simulink model "c00002M_harness"  (R2018a)
settings: Solver=ode3  StartTime=0.0  StopTime=10.0  RelTol=1e-3  EnableMultiTasking=on
undefined symbols (not defined in the file): b, DiscIntNeverNeededParam, J, K, L, PosMinimaW3, PosMinimaW4, R, sigbuilder_block
(part 1 of 75)
settings Model: Creator=aarrieta  LastModifiedBy=umarkiegi
settings DataIOCC: LimitDataPoints=on  SaveFormat=Array
settings OptimizationCC: LifeSpan=inf
settings DebuggingCC: UnderspecifiedInitializationDetection=Classic  MergeDetectMultiDrivingBlocksExec=none  SolverPrmCheckMsg=warning  StateNameClashWarn=warning  SFUnexpectedBacktrackingDiag=warning  SFNoUnconditionalDefaultTransitionDiag=warning  SFExecutionAtInitializationDiag=none
settings HardwareCC: ProdBitPerPointer=32  ProdBitPerSizeT=32  ProdBitPerPtrDiffT=32  ProdLargestAtomicFloat=None  ProdIntDivRoundTo=Undefined  ProdEndianess=Unspecified  ProdWordSize=32  ProdHWDeviceType=32-bit Generic
settings ModelReferenceCC: PropagateSignalLabelsOutOfModel=off
settings CodeAppCC: StateflowObjectComments=on
settings GRTTargetCC: TargetLangStandard=C89/C90 (ANSI)  GeneratePreprocessorConditionals=Disable all
settings ConfigComp: CovMetricSettings=dw  CovHtmlReporting=on  CovSaveCumulativeToWorkspaceVar=on  CovSaveSingleToWorkspaceVar=on  CovExternalEMLEnable=off  DVMaxTestCaseSteps=20  DVTestSuiteOptimization=CombinedObjectives (Nonlinear Extended)  DVDetectFloatOverflow=off

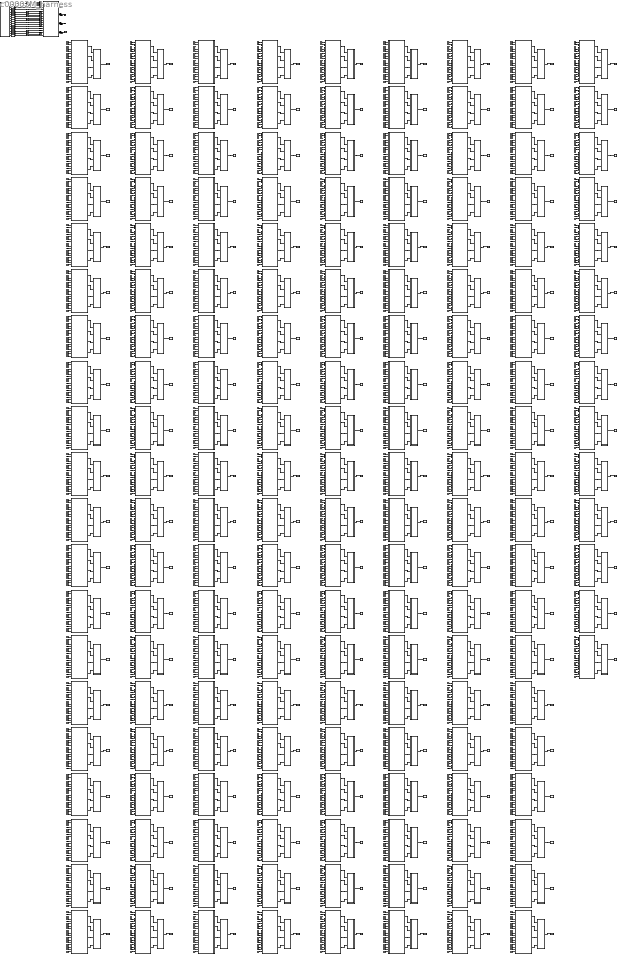
== system c00002M_harness ==
  CPSUT : Subsystem
  Eval : Subsystem
  Eval1 : Subsystem
  Eval10 : Subsystem
  Eval100 : Subsystem
  Eval101 : Subsystem
  Eval102 : Subsystem
  Eval103 : Subsystem
  Eval104 : Subsystem
  Eval105 : Subsystem
  Eval106 : Subsystem
  Eval107 : Subsystem
  Eval108 : Subsystem
  Eval109 : Subsystem
  Eval11 : Subsystem
  Eval110 : Subsystem
  Eval111 : Subsystem
  Eval112 : Subsystem
  Eval113 : Subsystem
  Eval114 : Subsystem
  Eval115 : Subsystem
  Eval116 : Subsystem
  Eval117 : Subsystem
  Eval118 : Subsystem
  Eval119 : Subsystem
  Eval12 : Subsystem
  Eval120 : Subsystem
  Eval121 : Subsystem
  Eval122 : Subsystem
  Eval123 : Subsystem
  Eval124 : Subsystem
  Eval125 : Subsystem
  Eval126 : Subsystem
  Eval127 : Subsystem
  Eval128 : Subsystem
  Eval129 : Subsystem
  Eval13 : Subsystem
  Eval130 : Subsystem
  Eval131 : Subsystem
  Eval132 : Subsystem
  Eval133 : Subsystem
  Eval134 : Subsystem
  Eval135 : Subsystem
  Eval136 : Subsystem
  Eval137 : Subsystem
  Eval138 : Subsystem
  Eval139 : Subsystem
  Eval14 : Subsystem
  Eval140 : Subsystem
  Eval141 : Subsystem
  Eval142 : Subsystem
  Eval143 : Subsystem
  Eval144 : Subsystem
  Eval145 : Subsystem
  Eval146 : Subsystem
  Eval147 : Subsystem
  Eval148 : Subsystem
  Eval149 : Subsystem
  Eval15 : Subsystem
  Eval150 : Subsystem
  Eval151 : Subsystem
  Eval152 : Subsystem
  Eval153 : Subsystem
  Eval154 : Subsystem
  Eval155 : Subsystem
  Eval156 : Subsystem
  Eval157 : Subsystem
  Eval158 : Subsystem
  Eval159 : Subsystem
  Eval16 : Subsystem
  Eval160 : Subsystem
  Eval161 : Subsystem
  Eval162 : Subsystem
  Eval163 : Subsystem
  Eval164 : Subsystem
  Eval165 : Subsystem
  Eval166 : Subsystem
  Eval167 : Subsystem
  Eval168 : Subsystem
  Eval169 : Subsystem
  Eval17 : Subsystem
  Eval170 : Subsystem
  Eval171 : Subsystem
  Eval172 : Subsystem
  Eval173 : Subsystem
  Eval18 : Subsystem
  Eval19 : Subsystem
  Eval2 : Subsystem
  Eval20 : Subsystem
  Eval21 : Subsystem
  Eval22 : Subsystem
  Eval23 : Subsystem
  Eval24 : Subsystem
  Eval25 : Subsystem
  Eval26 : Subsystem
  Eval27 : Subsystem
  Eval28 : Subsystem
  Eval29 : Subsystem
  Eval3 : Subsystem
  Eval30 : Subsystem
  Eval31 : Subsystem
  Eval32 : Subsystem
  Eval33 : Subsystem
  Eval34 : Subsystem
  Eval35 : Subsystem
  Eval36 : Subsystem
  Eval37 : Subsystem
  Eval38 : Subsystem
  Eval39 : Subsystem
  Eval4 : Subsystem
  Eval40 : Subsystem
  Eval41 : Subsystem
  Eval42 : Subsystem
  Eval43 : Subsystem
  Eval44 : Subsystem
  Eval45 : Subsystem
  Eval46 : Subsystem
  Eval47 : Subsystem
  Eval48 : Subsystem
  Eval49 : Subsystem
  Eval5 : Subsystem
  Eval50 : Subsystem
  Eval51 : Subsystem
  Eval52 : Subsystem
  Eval53 : Subsystem
  Eval54 : Subsystem
  Eval55 : Subsystem
  Eval56 : Subsystem
  Eval57 : Subsystem
  Eval58 : Subsystem
  Eval59 : Subsystem
  Eval6 : Subsystem
  Eval60 : Subsystem
  Eval61 : Subsystem
  Eval62 : Subsystem
  Eval63 : Subsystem
  Eval64 : Subsystem
  Eval65 : Subsystem
  Eval66 : Subsystem
  Eval67 : Subsystem
  Eval68 : Subsystem
  Eval69 : Subsystem
  Eval7 : Subsystem
  Eval70 : Subsystem
  Eval71 : Subsystem
  Eval72 : Subsystem
  Eval73 : Subsystem
  Eval74 : Subsystem
  Eval75 : Subsystem
  Eval76 : Subsystem
  Eval77 : Subsystem
  Eval78 : Subsystem
  Eval79 : Subsystem
  Eval8 : Subsystem
  Eval80 : Subsystem
  Eval81 : Subsystem
  Eval82 : Subsystem
  Eval83 : Subsystem
  Eval84 : Subsystem
  Eval85 : Subsystem
  Eval86 : Subsystem
  Eval87 : Subsystem
  Eval88 : Subsystem
  Eval89 : Subsystem
  Eval9 : Subsystem
  Eval90 : Subsystem
  Eval91 : Subsystem
  Eval92 : Subsystem
  Eval93 : Subsystem
  Eval94 : Subsystem
  Eval95 : Subsystem
  Eval96 : Subsystem
  Eval97 : Subsystem
  Eval98 : Subsystem
  Eval99 : Subsystem
  Inputs : Subsystem  Tag=STV Subsys  LoadFcn=sigbuilder_block('load');  StartFcn=sigbuilder_block('start');  StopFcn=sigbuilder_block('stop');  ClipboardFcn=sigbuilder_block('clipboard');  mask(Sigbuilder block){tuvar=[0:10]}
      mask init:
      | if ~strcmp(get_param(bdroot(gcb),'SimulationStatus'),'stopped'),tuvar = sigbuilder_block('maskInit'); end
      settings: CopyFcn=sigbuilder_block('copy');  DeleteFcn=sigbuilder_block('delete');  ModelCloseFcn=sigbuilder_block('modelClose');  PreSaveFcn=sigbuilder_block('preSave');  PauseFcn=sigbuilder_block('pause');  ContinueFcn=sigbuilder_block('continue');  NameChangeFcn=sigbuilder_block('namechange');  OpenFcn=sigbuilder_block('open');  CloseFcn=sigbuilder_block('close');
      mask Display: plot(0, 0, 100, 100,[2, 2, 32, 32, 2], [68, 8, 8, 68, 68],[32, 2], [38, 38], [32, 19, 2],[53, 60, 44], [32, 17, 17, 2],[16, 16, 31, 31]);txt = getActiveGroup(gcbh);text(2, 100, txt,'verticalAlignment', 'top');
  M001 : Subsystem
  M002 : Subsystem
  M003 : Subsystem
  M004 : Subsystem
  M005 : Subsystem
  M006 : Subsystem
  M007 : Subsystem
  M008 : Subsystem
  M009 : Subsystem
  M010 : Subsystem
  M011 : Subsystem
  M012 : Subsystem
  M013 : Subsystem
  M014 : Subsystem
  M015 : Subsystem
  M016 : Subsystem
  M017 : Subsystem
  M018 : Subsystem
  M019 : Subsystem
  M020 : Subsystem
  M021 : Subsystem
  M022 : Subsystem
  M023 : Subsystem
  M024 : Subsystem
  M025 : Subsystem
  M026 : Subsystem
  M027 : Subsystem
  M028 : Subsystem
  M029 : Subsystem
  M030 : Subsystem
  M031 : Subsystem
  M032 : Subsystem
  M033 : Subsystem
  M034 : Subsystem
  M035 : Subsystem
  M036 : Subsystem
  M037 : Subsystem
  M038 : Subsystem
  M039 : Subsystem
  M040 : Subsystem
  M041 : Subsystem
  M042 : Subsystem
  M043 : Subsystem
  M044 : Subsystem
  M045 : Subsystem
  M046 : Subsystem
  M047 : Subsystem
  M048 : Subsystem
  M049 : Subsystem
  M050 : Subsystem
  M051 : Subsystem
  M052 : Subsystem
  M053 : Subsystem
  M054 : Subsystem
  M055 : Subsystem
  M056 : Subsystem
  M057 : Subsystem
  M058 : Subsystem
  M059 : Subsystem
  M060 : Subsystem
  M061 : Subsystem
  M062 : Subsystem
  M063 : Subsystem
  M064 : Subsystem
  M065 : Subsystem
  M066 : Subsystem
  M067 : Subsystem
  M068 : Subsystem
  M069 : Subsystem
  M070 : Subsystem
  M071 : Subsystem
  M072 : Subsystem
  M073 : Subsystem
  M074 : Subsystem
  M075 : Subsystem
  M076 : Subsystem
  M077 : Subsystem
  M078 : Subsystem
  M079 : Subsystem
  M080 : Subsystem
  M081 : Subsystem
  M082 : Subsystem
  M083 : Subsystem
  M084 : Subsystem
  M085 : Subsystem
  M086 : Subsystem
  M087 : Subsystem
  M088 : Subsystem
  M089 : Subsystem
  M090 : Subsystem
  M091 : Subsystem
  M092 : Subsystem
  M093 : Subsystem
  M094 : Subsystem
  M095 : Subsystem
  M096 : Subsystem
  M097 : Subsystem
  M098 : Subsystem
  M099 : Subsystem
  M100 : Subsystem
  M101 : Subsystem
  M102 : Subsystem
  M103 : Subsystem
  M104 : Subsystem
  M105 : Subsystem
  M106 : Subsystem
  M107 : Subsystem
  M108 : Subsystem
  M109 : Subsystem
  M110 : Subsystem
  M111 : Subsystem
  M112 : Subsystem
  M113 : Subsystem
  M114 : Subsystem
  M115 : Subsystem
  M116 : Subsystem
  M117 : Subsystem
  M118 : Subsystem
  M119 : Subsystem
  M120 : Subsystem
  M121 : Subsystem
  M122 : Subsystem
  M123 : Subsystem
  M124 : Subsystem
  M125 : Subsystem
  M126 : Subsystem
  M127 : Subsystem
  M128 : Subsystem
  M129 : Subsystem
  M130 : Subsystem
  M131 : Subsystem
  M132 : Subsystem
  M133 : Subsystem
  M134 : Subsystem
  M135 : Subsystem
  M136 : Subsystem
  M137 : Subsystem
  M138 : Subsystem
  M139 : Subsystem
  M140 : Subsystem
  M141 : Subsystem
  M142 : Subsystem
  M143 : Subsystem
  M144 : Subsystem
  M145 : Subsystem
  M146 : Subsystem
  M147 : Subsystem
  M148 : Subsystem
  M149 : Subsystem
  M150 : Subsystem
  M151 : Subsystem
  M152 : Subsystem
  M153 : Subsystem
  M154 : Subsystem
  M155 : Subsystem
  M156 : Subsystem
  M157 : Subsystem
  M158 : Subsystem
  M159 : Subsystem
  M160 : Subsystem
  M161 : Subsystem
  M162 : Subsystem
  M163 : Subsystem
  M164 : Subsystem
  M165 : Subsystem
  M166 : Subsystem
  M167 : Subsystem
  M168 : Subsystem
  M169 : Subsystem
  M170 : Subsystem
  M171 : Subsystem
  M172 : Subsystem
  M173 : Subsystem
  M174 : Subsystem
  To Workspace : ToWorkspace  VariableName=mutant001  SampleTime=-1
  To Workspace1 : ToWorkspace  VariableName=mutant002  SampleTime=-1
  To Workspace10 : ToWorkspace  VariableName=mutant011  SampleTime=-1
  To Workspace100 : ToWorkspace  VariableName=mutant101  SampleTime=-1
  To Workspace101 : ToWorkspace  VariableName=mutant102  SampleTime=-1
  To Workspace102 : ToWorkspace  VariableName=mutant103  SampleTime=-1
  To Workspace103 : ToWorkspace  VariableName=mutant104  SampleTime=-1
  To Workspace104 : ToWorkspace  VariableName=mutant105  SampleTime=-1
  To Workspace105 : ToWorkspace  VariableName=mutant106  SampleTime=-1
  To Workspace106 : ToWorkspace  VariableName=mutant107  SampleTime=-1
  To Workspace107 : ToWorkspace  VariableName=mutant108  SampleTime=-1
  To Workspace108 : ToWorkspace  VariableName=mutant109  SampleTime=-1
  To Workspace109 : ToWorkspace  VariableName=mutant110  SampleTime=-1
  To Workspace11 : ToWorkspace  VariableName=mutant012  SampleTime=-1
  To Workspace110 : ToWorkspace  VariableName=mutant111  SampleTime=-1
  To Workspace111 : ToWorkspace  VariableName=mutant112  SampleTime=-1
  To Workspace112 : ToWorkspace  VariableName=mutant113  SampleTime=-1
  To Workspace113 : ToWorkspace  VariableName=mutant114  SampleTime=-1
  To Workspace114 : ToWorkspace  VariableName=mutant115  SampleTime=-1
  To Workspace115 : ToWorkspace  VariableName=mutant116  SampleTime=-1
  To Workspace116 : ToWorkspace  VariableName=mutant117  SampleTime=-1
  To Workspace117 : ToWorkspace  VariableName=mutant118  SampleTime=-1
  To Workspace118 : ToWorkspace  VariableName=mutant119  SampleTime=-1
  To Workspace119 : ToWorkspace  VariableName=mutant120  SampleTime=-1
  To Workspace12 : ToWorkspace  VariableName=mutant013  SampleTime=-1
  To Workspace120 : ToWorkspace  VariableName=mutant121  SampleTime=-1
  To Workspace121 : ToWorkspace  VariableName=mutant122  SampleTime=-1
  To Workspace122 : ToWorkspace  VariableName=mutant123  SampleTime=-1
  To Workspace123 : ToWorkspace  VariableName=mutant124  SampleTime=-1
  To Workspace124 : ToWorkspace  VariableName=mutant125  SampleTime=-1
  To Workspace125 : ToWorkspace  VariableName=mutant126  SampleTime=-1
  To Workspace126 : ToWorkspace  VariableName=mutant127  SampleTime=-1
  To Workspace127 : ToWorkspace  VariableName=mutant128  SampleTime=-1
  To Workspace128 : ToWorkspace  VariableName=mutant129  SampleTime=-1
  To Workspace129 : ToWorkspace  VariableName=mutant130  SampleTime=-1
  To Workspace13 : ToWorkspace  VariableName=mutant014  SampleTime=-1
  To Workspace130 : ToWorkspace  VariableName=mutant131  SampleTime=-1
  To Workspace131 : ToWorkspace  VariableName=mutant132  SampleTime=-1
  To Workspace132 : ToWorkspace  VariableName=mutant133  SampleTime=-1
  To Workspace133 : ToWorkspace  VariableName=mutant134  SampleTime=-1
  To Workspace134 : ToWorkspace  VariableName=mutant135  SampleTime=-1
  To Workspace135 : ToWorkspace  VariableName=mutant136  SampleTime=-1
  To Workspace136 : ToWorkspace  VariableName=mutant137  SampleTime=-1
  To Workspace137 : ToWorkspace  VariableName=mutant138  SampleTime=-1
  To Workspace138 : ToWorkspace  VariableName=mutant139  SampleTime=-1
  To Workspace139 : ToWorkspace  VariableName=mutant140  SampleTime=-1
  To Workspace14 : ToWorkspace  VariableName=mutant015  SampleTime=-1
  To Workspace140 : ToWorkspace  VariableName=mutant141  SampleTime=-1
  To Workspace141 : ToWorkspace  VariableName=mutant142  SampleTime=-1
  To Workspace142 : ToWorkspace  VariableName=mutant143  SampleTime=-1
  To Workspace143 : ToWorkspace  VariableName=mutant144  SampleTime=-1
  To Workspace144 : ToWorkspace  VariableName=mutant145  SampleTime=-1
  To Workspace145 : ToWorkspace  VariableName=mutant146  SampleTime=-1
  To Workspace146 : ToWorkspace  VariableName=mutant147  SampleTime=-1
  To Workspace147 : ToWorkspace  VariableName=mutant148  SampleTime=-1
  To Workspace148 : ToWorkspace  VariableName=mutant149  SampleTime=-1
  To Workspace149 : ToWorkspace  VariableName=mutant150  SampleTime=-1
  To Workspace15 : ToWorkspace  VariableName=mutant016  SampleTime=-1
  To Workspace150 : ToWorkspace  VariableName=mutant151  SampleTime=-1
  To Workspace151 : ToWorkspace  VariableName=mutant152  SampleTime=-1
  To Workspace152 : ToWorkspace  VariableName=mutant153  SampleTime=-1
  To Workspace153 : ToWorkspace  VariableName=mutant154  SampleTime=-1
  To Workspace154 : ToWorkspace  VariableName=mutant155  SampleTime=-1
  To Workspace155 : ToWorkspace  VariableName=mutant156  SampleTime=-1
  To Workspace156 : ToWorkspace  VariableName=mutant157  SampleTime=-1
  To Workspace157 : ToWorkspace  VariableName=mutant158  SampleTime=-1
  To Workspace158 : ToWorkspace  VariableName=mutant159  SampleTime=-1
  To Workspace159 : ToWorkspace  VariableName=mutant160  SampleTime=-1
  To Workspace16 : ToWorkspace  VariableName=mutant017  SampleTime=-1
  To Workspace160 : ToWorkspace  VariableName=mutant161  SampleTime=-1
  To Workspace161 : ToWorkspace  VariableName=mutant162  SampleTime=-1
  To Workspace162 : ToWorkspace  VariableName=mutant163  SampleTime=-1
  To Workspace163 : ToWorkspace  VariableName=mutant164  SampleTime=-1
  To Workspace164 : ToWorkspace  VariableName=mutant165  SampleTime=-1
  To Workspace165 : ToWorkspace  VariableName=mutant166  SampleTime=-1
  To Workspace166 : ToWorkspace  VariableName=mutant167  SampleTime=-1
  To Workspace167 : ToWorkspace  VariableName=mutant168  SampleTime=-1
  To Workspace168 : ToWorkspace  VariableName=mutant169  SampleTime=-1
  To Workspace169 : ToWorkspace  VariableName=mutant170  SampleTime=-1
  To Workspace17 : ToWorkspace  VariableName=mutant018  SampleTime=-1
  To Workspace170 : ToWorkspace  VariableName=mutant171  SampleTime=-1
  To Workspace171 : ToWorkspace  VariableName=mutant172  SampleTime=-1
  To Workspace172 : ToWorkspace  VariableName=mutant173  SampleTime=-1
  To Workspace173 : ToWorkspace  VariableName=mutant174  SampleTime=-1
  To Workspace18 : ToWorkspace  VariableName=mutant019  SampleTime=-1
  To Workspace19 : ToWorkspace  VariableName=mutant020  SampleTime=-1
  To Workspace2 : ToWorkspace  VariableName=mutant003  SampleTime=-1
  To Workspace20 : ToWorkspace  VariableName=mutant021  SampleTime=-1
  To Workspace21 : ToWorkspace  VariableName=mutant022  SampleTime=-1
  To Workspace22 : ToWorkspace  VariableName=mutant023  SampleTime=-1
  To Workspace23 : ToWorkspace  VariableName=mutant024  SampleTime=-1
  To Workspace24 : ToWorkspace  VariableName=mutant025  SampleTime=-1
  To Workspace25 : ToWorkspace  VariableName=mutant026  SampleTime=-1
  To Workspace26 : ToWorkspace  VariableName=mutant027  SampleTime=-1
  To Workspace27 : ToWorkspace  VariableName=mutant028  SampleTime=-1
  To Workspace28 : ToWorkspace  VariableName=mutant029  SampleTime=-1
  To Workspace29 : ToWorkspace  VariableName=mutant030  SampleTime=-1
  To Workspace3 : ToWorkspace  VariableName=mutant004  SampleTime=-1
  To Workspace30 : ToWorkspace  VariableName=mutant031  SampleTime=-1
  To Workspace31 : ToWorkspace  VariableName=mutant032  SampleTime=-1
  To Workspace32 : ToWorkspace  VariableName=mutant033  SampleTime=-1
  To Workspace33 : ToWorkspace  VariableName=mutant034  SampleTime=-1
  To Workspace34 : ToWorkspace  VariableName=mutant035  SampleTime=-1
  To Workspace35 : ToWorkspace  VariableName=mutant036  SampleTime=-1
  To Workspace36 : ToWorkspace  VariableName=mutant037  SampleTime=-1
  To Workspace37 : ToWorkspace  VariableName=mutant038  SampleTime=-1
  To Workspace38 : ToWorkspace  VariableName=mutant039  SampleTime=-1
  To Workspace39 : ToWorkspace  VariableName=mutant040  SampleTime=-1
  To Workspace4 : ToWorkspace  VariableName=mutant005  SampleTime=-1
  To Workspace40 : ToWorkspace  VariableName=mutant041  SampleTime=-1
  To Workspace41 : ToWorkspace  VariableName=mutant042  SampleTime=-1
  To Workspace42 : ToWorkspace  VariableName=mutant043  SampleTime=-1
  To Workspace43 : ToWorkspace  VariableName=mutant044  SampleTime=-1
  To Workspace44 : ToWorkspace  VariableName=mutant045  SampleTime=-1
  To Workspace45 : ToWorkspace  VariableName=mutant046  SampleTime=-1
  To Workspace46 : ToWorkspace  VariableName=mutant047  SampleTime=-1
  To Workspace47 : ToWorkspace  VariableName=mutant048  SampleTime=-1
  To Workspace48 : ToWorkspace  VariableName=mutant049  SampleTime=-1
  To Workspace49 : ToWorkspace  VariableName=mutant050  SampleTime=-1
  To Workspace5 : ToWorkspace  VariableName=mutant006  SampleTime=-1
  To Workspace50 : ToWorkspace  VariableName=mutant051  SampleTime=-1
  To Workspace51 : ToWorkspace  VariableName=mutant052  SampleTime=-1
  To Workspace52 : ToWorkspace  VariableName=mutant053  SampleTime=-1
  To Workspace53 : ToWorkspace  VariableName=mutant054  SampleTime=-1
  To Workspace54 : ToWorkspace  VariableName=mutant055  SampleTime=-1
  To Workspace55 : ToWorkspace  VariableName=mutant056  SampleTime=-1
  To Workspace56 : ToWorkspace  VariableName=mutant057  SampleTime=-1
  To Workspace57 : ToWorkspace  VariableName=mutant058  SampleTime=-1
  To Workspace58 : ToWorkspace  VariableName=mutant059  SampleTime=-1
  To Workspace59 : ToWorkspace  VariableName=mutant060  SampleTime=-1
  To Workspace6 : ToWorkspace  VariableName=mutant007  SampleTime=-1
  To Workspace60 : ToWorkspace  VariableName=mutant061  SampleTime=-1
  To Workspace61 : ToWorkspace  VariableName=mutant062  SampleTime=-1
  To Workspace62 : ToWorkspace  VariableName=mutant063  SampleTime=-1
  To Workspace63 : ToWorkspace  VariableName=mutant064  SampleTime=-1
  To Workspace64 : ToWorkspace  VariableName=mutant065  SampleTime=-1
  To Workspace65 : ToWorkspace  VariableName=mutant066  SampleTime=-1
  To Workspace66 : ToWorkspace  VariableName=mutant067  SampleTime=-1
  To Workspace67 : ToWorkspace  VariableName=mutant068  SampleTime=-1
  To Workspace68 : ToWorkspace  VariableName=mutant069  SampleTime=-1
  To Workspace69 : ToWorkspace  VariableName=mutant070  SampleTime=-1
  To Workspace7 : ToWorkspace  VariableName=mutant008  SampleTime=-1
  To Workspace70 : ToWorkspace  VariableName=mutant071  SampleTime=-1
  To Workspace71 : ToWorkspace  VariableName=mutant072  SampleTime=-1
  To Workspace72 : ToWorkspace  VariableName=mutant073  SampleTime=-1
  To Workspace73 : ToWorkspace  VariableName=mutant074  SampleTime=-1
  To Workspace74 : ToWorkspace  VariableName=mutant075  SampleTime=-1
  To Workspace75 : ToWorkspace  VariableName=mutant076  SampleTime=-1
  To Workspace76 : ToWorkspace  VariableName=mutant077  SampleTime=-1
  To Workspace77 : ToWorkspace  VariableName=mutant078  SampleTime=-1
  To Workspace78 : ToWorkspace  VariableName=mutant079  SampleTime=-1
  To Workspace79 : ToWorkspace  VariableName=mutant080  SampleTime=-1
  To Workspace8 : ToWorkspace  VariableName=mutant009  SampleTime=-1
  To Workspace80 : ToWorkspace  VariableName=mutant081  SampleTime=-1
  To Workspace81 : ToWorkspace  VariableName=mutant082  SampleTime=-1
  To Workspace82 : ToWorkspace  VariableName=mutant083  SampleTime=-1
  To Workspace83 : ToWorkspace  VariableName=mutant084  SampleTime=-1
  To Workspace84 : ToWorkspace  VariableName=mutant085  SampleTime=-1
  To Workspace85 : ToWorkspace  VariableName=mutant086  SampleTime=-1
  To Workspace86 : ToWorkspace  VariableName=mutant087  SampleTime=-1
  To Workspace87 : ToWorkspace  VariableName=mutant088  SampleTime=-1
  To Workspace88 : ToWorkspace  VariableName=mutant089  SampleTime=-1
  To Workspace89 : ToWorkspace  VariableName=mutant090  SampleTime=-1
  To Workspace9 : ToWorkspace  VariableName=mutant010  SampleTime=-1
  To Workspace90 : ToWorkspace  VariableName=mutant091  SampleTime=-1
  To Workspace91 : ToWorkspace  VariableName=mutant092  SampleTime=-1
  To Workspace92 : ToWorkspace  VariableName=mutant093  SampleTime=-1
  To Workspace93 : ToWorkspace  VariableName=mutant094  SampleTime=-1
  To Workspace94 : ToWorkspace  VariableName=mutant095  SampleTime=-1
  To Workspace95 : ToWorkspace  VariableName=mutant096  SampleTime=-1
  To Workspace96 : ToWorkspace  VariableName=mutant097  SampleTime=-1
  To Workspace97 : ToWorkspace  VariableName=mutant098  SampleTime=-1
  To Workspace98 : ToWorkspace  VariableName=mutant099  SampleTime=-1
  To Workspace99 : ToWorkspace  VariableName=mutant100  SampleTime=-1
  dtc_CW1C : DataTypeConversion
  dtc_CW2C : DataTypeConversion
  dtc_CW3C : DataTypeConversion
  dtc_CW4C : DataTypeConversion
  dtc_DW1 : DataTypeConversion
  dtc_DW2 : DataTypeConversion
  dtc_DW4 : DataTypeConversion
  dtc_LD : DataTypeConversion
  dtc_O{1..4} (4 alike) : DataTypeConversion
  dtc_P1W2 : DataTypeConversion
  dtc_P1W3 : DataTypeConversion
  dtc_P2W3 : DataTypeConversion
  dtc_P3W4 : DataTypeConversion
  W1Pos : Outport
  W2Pos : Outport  Port=2
  W3Pos : Outport  Port=3
  W4Pos : Outport  Port=4
  tag scope: out1=global, out2=global, out3=global, out4=global
  wires:
  CPSUT/2(W2Pos) -> [out2], W2Pos/1
  CPSUT/3(W3Pos) -> W3Pos/1, [out3]
  CPSUT/4(W4Pos) -> W4Pos/1, [out4]
  [in1] -> M001/1(DW1)
  [in2] -> M001/2(DW2)
  [in4] -> M001/3(DW4)
  [in5] -> M001/4(P1W2)
  [in6] -> M001/5(P2W3)
  [in7] -> M001/6(P1W3)
  [in8] -> M001/7(P3W4)
  [in10] -> M001/8(O1)
  [in11] -> M001/9(O2)
  [in12] -> M001/10(O3)
  [in13] -> M001/11(O4)
  [in14] -> M001/12(LD)
  [in15] -> M001/13(CW1C)
  [in16] -> M001/14(CW2C)
  [in17] -> M001/15(CW3C)
  [in18] -> M001/16(CW4C)
  CPSUT/1(W1Pos) -> [out1], W1Pos/1
  M001/1(W1Pos) -> Eval/1(In1)
  M001/2(W2Pos) -> Eval/2(In2)
  M001/3(W3Pos) -> Eval/3(In3)
  M001/4(W4Pos) -> Eval/4(In4)
  Eval/1(Out1) -> To Workspace/1
  [in1] -> M002/1(DW1)
  [in2] -> M002/2(DW2)
  [in4] -> M002/3(DW4)
  [in5] -> M002/4(P1W2)
  [in6] -> M002/5(P2W3)
  [in7] -> M002/6(P1W3)
  [in8] -> M002/7(P3W4)
  [in10] -> M002/8(O1)
  [in11] -> M002/9(O2)
  [in12] -> M002/10(O3)
  [in13] -> M002/11(O4)
  [in14] -> M002/12(LD)
  [in15] -> M002/13(CW1C)
  [in16] -> M002/14(CW2C)
  [in17] -> M002/15(CW3C)
  [in18] -> M002/16(CW4C)
  M002/1(W1Pos) -> Eval1/1(In1)
  M002/2(W2Pos) -> Eval1/2(In2)
  M002/3(W3Pos) -> Eval1/3(In3)
  M002/4(W4Pos) -> Eval1/4(In4)
  Eval1/1(Out1) -> To Workspace1/1
  [in1] -> M003/1(DW1)
  [in2] -> M003/2(DW2)
  [in4] -> M003/3(DW4)
  [in5] -> M003/4(P1W2)
  [in6] -> M003/5(P2W3)
  [in7] -> M003/6(P1W3)
  [in8] -> M003/7(P3W4)
  [in10] -> M003/8(O1)
  [in11] -> M003/9(O2)
  [in12] -> M003/10(O3)
  [in13] -> M003/11(O4)
  [in14] -> M003/12(LD)
  [in15] -> M003/13(CW1C)
  [in16] -> M003/14(CW2C)
  [in17] -> M003/15(CW3C)
  [in18] -> M003/16(CW4C)
  M003/1(W1Pos) -> Eval2/1(In1)
  M003/2(W2Pos) -> Eval2/2(In2)
  M003/3(W3Pos) -> Eval2/3(In3)
  M003/4(W4Pos) -> Eval2/4(In4)
  Eval2/1(Out1) -> To Workspace2/1
  [in1] -> M004/1(DW1)
  [in2] -> M004/2(DW2)
  [in4] -> M004/3(DW4)
  [in5] -> M004/4(P1W2)
  [in6] -> M004/5(P2W3)
  [in7] -> M004/6(P1W3)
  [in8] -> M004/7(P3W4)
  [in10] -> M004/8(O1)
  [in11] -> M004/9(O2)
  [in12] -> M004/10(O3)
  [in13] -> M004/11(O4)
  [in14] -> M004/12(LD)
  [in15] -> M004/13(CW1C)
  [in16] -> M004/14(CW2C)
  [in17] -> M004/15(CW3C)
  [in18] -> M004/16(CW4C)
  M004/1(W1Pos) -> Eval3/1(In1)
  M004/2(W2Pos) -> Eval3/2(In2)
  M004/3(W3Pos) -> Eval3/3(In3)
  M004/4(W4Pos) -> Eval3/4(In4)
  Eval3/1(Out1) -> To Workspace3/1
  [in1] -> M005/1(DW1)
  [in2] -> M005/2(DW2)
  [in4] -> M005/3(DW4)
  [in5] -> M005/4(P1W2)
  [in6] -> M005/5(P2W3)
  [in7] -> M005/6(P1W3)
  [in8] -> M005/7(P3W4)
  [in10] -> M005/8(O1)
  [in11] -> M005/9(O2)
  [in12] -> M005/10(O3)
  [in13] -> M005/11(O4)
  [in14] -> M005/12(LD)
  [in15] -> M005/13(CW1C)
  [in16] -> M005/14(CW2C)
  [in17] -> M005/15(CW3C)
  [in18] -> M005/16(CW4C)
  M005/1(W1Pos) -> Eval4/1(In1)
  M005/2(W2Pos) -> Eval4/2(In2)
  M005/3(W3Pos) -> Eval4/3(In3)
  M005/4(W4Pos) -> Eval4/4(In4)
  Eval4/1(Out1) -> To Workspace4/1
  [in1] -> M006/1(DW1)
  [in2] -> M006/2(DW2)
  [in4] -> M006/3(DW4)
  [in5] -> M006/4(P1W2)
  [in6] -> M006/5(P2W3)
  [in7] -> M006/6(P1W3)
  [in8] -> M006/7(P3W4)
  [in10] -> M006/8(O1)
  [in11] -> M006/9(O2)
  [in12] -> M006/10(O3)
  [in13] -> M006/11(O4)
  [in14] -> M006/12(LD)
  [in15] -> M006/13(CW1C)
  [in16] -> M006/14(CW2C)
  [in17] -> M006/15(CW3C)
  [in18] -> M006/16(CW4C)
  M006/1(W1Pos) -> Eval5/1(In1)
  M006/2(W2Pos) -> Eval5/2(In2)
  M006/3(W3Pos) -> Eval5/3(In3)
  M006/4(W4Pos) -> Eval5/4(In4)
  Eval5/1(Out1) -> To Workspace5/1
  [in1] -> M007/1(DW1)
  [in2] -> M007/2(DW2)
  [in4] -> M007/3(DW4)
  [in5] -> M007/4(P1W2)
  [in6] -> M007/5(P2W3)
  [in7] -> M007/6(P1W3)
  [in8] -> M007/7(P3W4)
  [in10] -> M007/8(O1)
  [in11] -> M007/9(O2)
  [in12] -> M007/10(O3)
  [in13] -> M007/11(O4)
  [in14] -> M007/12(LD)
  [in15] -> M007/13(CW1C)
  [in16] -> M007/14(CW2C)
  [in17] -> M007/15(CW3C)
  [in18] -> M007/16(CW4C)
  M007/1(W1Pos) -> Eval6/1(In1)
  M007/2(W2Pos) -> Eval6/2(In2)
  M007/3(W3Pos) -> Eval6/3(In3)
  M007/4(W4Pos) -> Eval6/4(In4)
  Eval6/1(Out1) -> To Workspace6/1
  [in1] -> M008/1(DW1)
  [in2] -> M008/2(DW2)
  [in4] -> M008/3(DW4)
  [in5] -> M008/4(P1W2)
  [in6] -> M008/5(P2W3)
  [in7] -> M008/6(P1W3)
  [in8] -> M008/7(P3W4)
  [in10] -> M008/8(O1)
  [in11] -> M008/9(O2)
  [in12] -> M008/10(O3)
  [in13] -> M008/11(O4)
  [in14] -> M008/12(LD)
  [in15] -> M008/13(CW1C)
  [in16] -> M008/14(CW2C)
  [in17] -> M008/15(CW3C)
  [in18] -> M008/16(CW4C)
  M008/1(W1Pos) -> Eval7/1(In1)
  M008/2(W2Pos) -> Eval7/2(In2)
  M008/3(W3Pos) -> Eval7/3(In3)
  M008/4(W4Pos) -> Eval7/4(In4)
  Eval7/1(Out1) -> To Workspace7/1
  [in1] -> M009/1(DW1)
  [in2] -> M009/2(DW2)
  [in4] -> M009/3(DW4)
  [in5] -> M009/4(P1W2)
  [in6] -> M009/5(P2W3)
  [in7] -> M009/6(P1W3)
  [in8] -> M009/7(P3W4)
  [in10] -> M009/8(O1)
  [in11] -> M009/9(O2)
  [in12] -> M009/10(O3)
  [in13] -> M009/11(O4)
  [in14] -> M009/12(LD)
  [in15] -> M009/13(CW1C)
  [in16] -> M009/14(CW2C)
  [in17] -> M009/15(CW3C)
  [in18] -> M009/16(CW4C)
  M009/1(W1Pos) -> Eval8/1(In1)
  M009/2(W2Pos) -> Eval8/2(In2)
  M009/3(W3Pos) -> Eval8/3(In3)
  M009/4(W4Pos) -> Eval8/4(In4)
  Eval8/1(Out1) -> To Workspace8/1
  [in1] -> M010/1(DW1)
  [in2] -> M010/2(DW2)
  [in4] -> M010/3(DW4)
  [in5] -> M010/4(P1W2)
  [in6] -> M010/5(P2W3)
  [in7] -> M010/6(P1W3)
  [in8] -> M010/7(P3W4)
  [in10] -> M010/8(O1)
  [in11] -> M010/9(O2)
  [in12] -> M010/10(O3)
  [in13] -> M010/11(O4)
  [in14] -> M010/12(LD)
  [in15] -> M010/13(CW1C)
  [in16] -> M010/14(CW2C)
  [in17] -> M010/15(CW3C)
  [in18] -> M010/16(CW4C)
  M010/1(W1Pos) -> Eval9/1(In1)
  M010/2(W2Pos) -> Eval9/2(In2)
  M010/3(W3Pos) -> Eval9/3(In3)
  M010/4(W4Pos) -> Eval9/4(In4)
  Eval9/1(Out1) -> To Workspace9/1
  [in1] -> M011/1(DW1)
  [in2] -> M011/2(DW2)
  [in4] -> M011/3(DW4)
  [in5] -> M011/4(P1W2)
  [in6] -> M011/5(P2W3)
  [in7] -> M011/6(P1W3)
  [in8] -> M011/7(P3W4)
  [in10] -> M011/8(O1)
  [in11] -> M011/9(O2)
  [in12] -> M011/10(O3)
  [in13] -> M011/11(O4)
  [in14] -> M011/12(LD)
  [in15] -> M011/13(CW1C)
  [in16] -> M011/14(CW2C)
  [in17] -> M011/15(CW3C)
  [in18] -> M011/16(CW4C)
  M011/1(W1Pos) -> Eval10/1(In1)
  M011/2(W2Pos) -> Eval10/2(In2)
  M011/3(W3Pos) -> Eval10/3(In3)
  M011/4(W4Pos) -> Eval10/4(In4)
  Eval10/1(Out1) -> To Workspace10/1
  [in1] -> M012/1(DW1)
  [in2] -> M012/2(DW2)
  [in4] -> M012/3(DW4)
  [in5] -> M012/4(P1W2)
  [in6] -> M012/5(P2W3)
  [in7] -> M012/6(P1W3)
  [in8] -> M012/7(P3W4)
  [in10] -> M012/8(O1)
  [in11] -> M012/9(O2)
  [in12] -> M012/10(O3)
  [in13] -> M012/11(O4)
  [in14] -> M012/12(LD)
  [in15] -> M012/13(CW1C)
  [in16] -> M012/14(CW2C)
  [in17] -> M012/15(CW3C)
  [in18] -> M012/16(CW4C)
  M012/1(W1Pos) -> Eval11/1(In1)
  M012/2(W2Pos) -> Eval11/2(In2)
  M012/3(W3Pos) -> Eval11/3(In3)
  M012/4(W4Pos) -> Eval11/4(In4)
  Eval11/1(Out1) -> To Workspace11/1
  [in1] -> M013/1(DW1)
  [in2] -> M013/2(DW2)
  [in4] -> M013/3(DW4)
  [in5] -> M013/4(P1W2)
  [in6] -> M013/5(P2W3)
  [in7] -> M013/6(P1W3)
  [in8] -> M013/7(P3W4)
  [in10] -> M013/8(O1)
  [in11] -> M013/9(O2)
  [in12] -> M013/10(O3)
  [in13] -> M013/11(O4)
  [in14] -> M013/12(LD)
  [in15] -> M013/13(CW1C)
  [in16] -> M013/14(CW2C)
  [in17] -> M013/15(CW3C)
  [in18] -> M013/16(CW4C)
  M013/1(W1Pos) -> Eval12/1(In1)
  M013/2(W2Pos) -> Eval12/2(In2)
  M013/3(W3Pos) -> Eval12/3(In3)
  M013/4(W4Pos) -> Eval12/4(In4)
  Eval12/1(Out1) -> To Workspace12/1
  [in1] -> M014/1(DW1)
  [in2] -> M014/2(DW2)
  [in4] -> M014/3(DW4)
  [in5] -> M014/4(P1W2)
  [in6] -> M014/5(P2W3)
  [in7] -> M014/6(P1W3)
  [in8] -> M014/7(P3W4)
  [in10] -> M014/8(O1)
  [in11] -> M014/9(O2)
  [in12] -> M014/10(O3)
  [in13] -> M014/11(O4)
  [in14] -> M014/12(LD)
  [in15] -> M014/13(CW1C)
  [in16] -> M014/14(CW2C)
  [in17] -> M014/15(CW3C)
  [in18] -> M014/16(CW4C)
  M014/1(W1Pos) -> Eval13/1(In1)
  M014/2(W2Pos) -> Eval13/2(In2)
  M014/3(W3Pos) -> Eval13/3(In3)
  M014/4(W4Pos) -> Eval13/4(In4)
  Eval13/1(Out1) -> To Workspace13/1
  [in1] -> M015/1(DW1)
  [in2] -> M015/2(DW2)
  [in4] -> M015/3(DW4)
  [in5] -> M015/4(P1W2)
  [in6] -> M015/5(P2W3)
  [in7] -> M015/6(P1W3)
  [in8] -> M015/7(P3W4)
  [in10] -> M015/8(O1)
  [in11] -> M015/9(O2)
  [in12] -> M015/10(O3)
  [in13] -> M015/11(O4)
  [in14] -> M015/12(LD)
  [in15] -> M015/13(CW1C)
  [in16] -> M015/14(CW2C)
  [in17] -> M015/15(CW3C)
  [in18] -> M015/16(CW4C)
  M015/1(W1Pos) -> Eval14/1(In1)
  M015/2(W2Pos) -> Eval14/2(In2)
  M015/3(W3Pos) -> Eval14/3(In3)
  M015/4(W4Pos) -> Eval14/4(In4)
  Eval14/1(Out1) -> To Workspace14/1
  [in1] -> M016/1(DW1)
  [in2] -> M016/2(DW2)
  [in4] -> M016/3(DW4)
  [in5] -> M016/4(P1W2)
  [in6] -> M016/5(P2W3)
  [in7] -> M016/6(P1W3)
  [in8] -> M016/7(P3W4)
  [in10] -> M016/8(O1)
  [in11] -> M016/9(O2)
  [in12] -> M016/10(O3)
  [in13] -> M016/11(O4)
  [in14] -> M016/12(LD)
  [in15] -> M016/13(CW1C)
  [in16] -> M016/14(CW2C)
  [in17] -> M016/15(CW3C)
  [in18] -> M016/16(CW4C)
  M016/1(W1Pos) -> Eval15/1(In1)
  M016/2(W2Pos) -> Eval15/2(In2)
  M016/3(W3Pos) -> Eval15/3(In3)
  M016/4(W4Pos) -> Eval15/4(In4)
  Eval15/1(Out1) -> To Workspace15/1
  [in1] -> M017/1(DW1)
  [in2] -> M017/2(DW2)
  [in4] -> M017/3(DW4)
  [in5] -> M017/4(P1W2)
  [in6] -> M017/5(P2W3)
  [in7] -> M017/6(P1W3)
  [in8] -> M017/7(P3W4)
  [in10] -> M017/8(O1)
  [in11] -> M017/9(O2)
  [in12] -> M017/10(O3)
  [in13] -> M017/11(O4)
  [in14] -> M017/12(LD)
  [in15] -> M017/13(CW1C)
  [in16] -> M017/14(CW2C)
  [in17] -> M017/15(CW3C)
  [in18] -> M017/16(CW4C)
  M017/1(W1Pos) -> Eval16/1(In1)
  M017/2(W2Pos) -> Eval16/2(In2)
  M017/3(W3Pos) -> Eval16/3(In3)
  M017/4(W4Pos) -> Eval16/4(In4)
  Eval16/1(Out1) -> To Workspace16/1
  [in1] -> M018/1(DW1)
  [in2] -> M018/2(DW2)
  [in4] -> M018/3(DW4)
  [in5] -> M018/4(P1W2)
  [in6] -> M018/5(P2W3)
  [in7] -> M018/6(P1W3)
  [in8] -> M018/7(P3W4)
  [in10] -> M018/8(O1)
  [in11] -> M018/9(O2)
  [in12] -> M018/10(O3)
  [in13] -> M018/11(O4)
  [in14] -> M018/12(LD)
  [in15] -> M018/13(CW1C)
  [in16] -> M018/14(CW2C)
  [in17] -> M018/15(CW3C)
  [in18] -> M018/16(CW4C)
  M018/1(W1Pos) -> Eval17/1(In1)
  M018/2(W2Pos) -> Eval17/2(In2)
  M018/3(W3Pos) -> Eval17/3(In3)
  M018/4(W4Pos) -> Eval17/4(In4)
  Eval17/1(Out1) -> To Workspace17/1
  [in1] -> M019/1(DW1)
  [in2] -> M019/2(DW2)
  [in4] -> M019/3(DW4)
  [in5] -> M019/4(P1W2)
  [in6] -> M019/5(P2W3)
  [in7] -> M019/6(P1W3)
  [in8] -> M019/7(P3W4)
  [in10] -> M019/8(O1)
  [in11] -> M019/9(O2)
  [in12] -> M019/10(O3)
  [in13] -> M019/11(O4)
  [in14] -> M019/12(LD)
  [in15] -> M019/13(CW1C)
  [in16] -> M019/14(CW2C)
  [in17] -> M019/15(CW3C)
  [in18] -> M019/16(CW4C)
  M019/1(W1Pos) -> Eval18/1(In1)
  M019/2(W2Pos) -> Eval18/2(In2)
  M019/3(W3Pos) -> Eval18/3(In3)
  M019/4(W4Pos) -> Eval18/4(In4)
  Eval18/1(Out1) -> To Workspace18/1
  [in1] -> M020/1(DW1)
  [in2] -> M020/2(DW2)
  [in4] -> M020/3(DW4)
  [in5] -> M020/4(P1W2)
  [in6] -> M020/5(P2W3)
  [in7] -> M020/6(P1W3)
  [in8] -> M020/7(P3W4)
  [in10] -> M020/8(O1)
  [in11] -> M020/9(O2)
  [in12] -> M020/10(O3)
  [in13] -> M020/11(O4)
  [in14] -> M020/12(LD)
  [in15] -> M020/13(CW1C)
  [in16] -> M020/14(CW2C)
  [in17] -> M020/15(CW3C)
  [in18] -> M020/16(CW4C)
  M020/1(W1Pos) -> Eval19/1(In1)
  M020/2(W2Pos) -> Eval19/2(In2)
  M020/3(W3Pos) -> Eval19/3(In3)
  M020/4(W4Pos) -> Eval19/4(In4)
  Eval19/1(Out1) -> To Workspace19/1
  [in1] -> M021/1(DW1)
  [in2] -> M021/2(DW2)
  [in4] -> M021/3(DW4)
  [in5] -> M021/4(P1W2)
  [in6] -> M021/5(P2W3)
  [in7] -> M021/6(P1W3)
  [in8] -> M021/7(P3W4)
  [in10] -> M021/8(O1)
  [in11] -> M021/9(O2)
  [in12] -> M021/10(O3)
  [in13] -> M021/11(O4)
  [in14] -> M021/12(LD)
  [in15] -> M021/13(CW1C)
  [in16] -> M021/14(CW2C)
  [in17] -> M021/15(CW3C)
  [in18] -> M021/16(CW4C)
  M021/1(W1Pos) -> Eval20/1(In1)
  M021/2(W2Pos) -> Eval20/2(In2)
  M021/3(W3Pos) -> Eval20/3(In3)
  M021/4(W4Pos) -> Eval20/4(In4)
  Eval20/1(Out1) -> To Workspace20/1
  [in1] -> M022/1(DW1)
  [in2] -> M022/2(DW2)
  [in4] -> M022/3(DW4)
  [in5] -> M022/4(P1W2)
  [in6] -> M022/5(P2W3)
  [in7] -> M022/6(P1W3)
  [in8] -> M022/7(P3W4)
  [in10] -> M022/8(O1)
  [in11] -> M022/9(O2)
  [in12] -> M022/10(O3)
  [in13] -> M022/11(O4)
  [in14] -> M022/12(LD)
  [in15] -> M022/13(CW1C)
  [in16] -> M022/14(CW2C)
  [in17] -> M022/15(CW3C)
  [in18] -> M022/16(CW4C)
  M022/1(W1Pos) -> Eval21/1(In1)
  M022/2(W2Pos) -> Eval21/2(In2)
  M022/3(W3Pos) -> Eval21/3(In3)
  M022/4(W4Pos) -> Eval21/4(In4)
  Eval21/1(Out1) -> To Workspace21/1
  [in1] -> M023/1(DW1)
  [in2] -> M023/2(DW2)
  [in4] -> M023/3(DW4)
  [in5] -> M023/4(P1W2)
  [in6] -> M023/5(P2W3)
  [in7] -> M023/6(P1W3)
  [in8] -> M023/7(P3W4)
  [in10] -> M023/8(O1)
  [in11] -> M023/9(O2)
  [in12] -> M023/10(O3)
  [in13] -> M023/11(O4)
  [in14] -> M023/12(LD)
  [in15] -> M023/13(CW1C)
  [in16] -> M023/14(CW2C)
  [in17] -> M023/15(CW3C)
  [in18] -> M023/16(CW4C)
  M023/1(W1Pos) -> Eval22/1(In1)
  M023/2(W2Pos) -> Eval22/2(In2)
  M023/3(W3Pos) -> Eval22/3(In3)
  M023/4(W4Pos) -> Eval22/4(In4)
  Eval22/1(Out1) -> To Workspace22/1
  [in1] -> M024/1(DW1)
  [in2] -> M024/2(DW2)
  [in4] -> M024/3(DW4)
  [in5] -> M024/4(P1W2)
  [in6] -> M024/5(P2W3)
  [in7] -> M024/6(P1W3)
  [in8] -> M024/7(P3W4)
  [in10] -> M024/8(O1)
  [in11] -> M024/9(O2)
  [in12] -> M024/10(O3)
  [in13] -> M024/11(O4)
  [in14] -> M024/12(LD)
  [in15] -> M024/13(CW1C)
  [in16] -> M024/14(CW2C)
  [in17] -> M024/15(CW3C)
  [in18] -> M024/16(CW4C)
  M024/1(W1Pos) -> Eval23/1(In1)
  M024/2(W2Pos) -> Eval23/2(In2)
  M024/3(W3Pos) -> Eval23/3(In3)
  M024/4(W4Pos) -> Eval23/4(In4)
  Eval23/1(Out1) -> To Workspace23/1
  [in1] -> M025/1(DW1)
  [in2] -> M025/2(DW2)
  [in4] -> M025/3(DW4)
  [in5] -> M025/4(P1W2)
  [in6] -> M025/5(P2W3)
  [in7] -> M025/6(P1W3)
  [in8] -> M025/7(P3W4)
  [in10] -> M025/8(O1)
  [in11] -> M025/9(O2)
  [in12] -> M025/10(O3)
  [in13] -> M025/11(O4)
  [in14] -> M025/12(LD)
  [in15] -> M025/13(CW1C)
  [in16] -> M025/14(CW2C)
  [in17] -> M025/15(CW3C)
  [in18] -> M025/16(CW4C)
  M025/1(W1Pos) -> Eval24/1(In1)
  M025/2(W2Pos) -> Eval24/2(In2)
  M025/3(W3Pos) -> Eval24/3(In3)
  M025/4(W4Pos) -> Eval24/4(In4)
  Eval24/1(Out1) -> To Workspace24/1
  [in1] -> M026/1(DW1)
  [in2] -> M026/2(DW2)
  [in4] -> M026/3(DW4)
  [in5] -> M026/4(P1W2)
  [in6] -> M026/5(P2W3)
  [in7] -> M026/6(P1W3)
  [in8] -> M026/7(P3W4)
  [in10] -> M026/8(O1)
  [in11] -> M026/9(O2)
  [in12] -> M026/10(O3)
  [in13] -> M026/11(O4)
  [in14] -> M026/12(LD)
  [in15] -> M026/13(CW1C)
  [in16] -> M026/14(CW2C)
  [in17] -> M026/15(CW3C)
  [in18] -> M026/16(CW4C)
  M026/1(W1Pos) -> Eval25/1(In1)
  M026/2(W2Pos) -> Eval25/2(In2)
  M026/3(W3Pos) -> Eval25/3(In3)
  M026/4(W4Pos) -> Eval25/4(In4)
  Eval25/1(Out1) -> To Workspace25/1
  [in1] -> M027/1(DW1)
  [in2] -> M027/2(DW2)
  [in4] -> M027/3(DW4)
  [in5] -> M027/4(P1W2)
  [in6] -> M027/5(P2W3)
  [in7] -> M027/6(P1W3)
  [in8] -> M027/7(P3W4)
  [in10] -> M027/8(O1)
  [in11] -> M027/9(O2)
  [in12] -> M027/10(O3)
  [in13] -> M027/11(O4)
  [in14] -> M027/12(LD)
  [in15] -> M027/13(CW1C)
  [in16] -> M027/14(CW2C)
  [in17] -> M027/15(CW3C)
  [in18] -> M027/16(CW4C)
  M027/1(W1Pos) -> Eval26/1(In1)
  M027/2(W2Pos) -> Eval26/2(In2)
  M027/3(W3Pos) -> Eval26/3(In3)
  M027/4(W4Pos) -> Eval26/4(In4)
  Eval26/1(Out1) -> To Workspace26/1
  [in1] -> M028/1(DW1)
  [in2] -> M028/2(DW2)
  [in4] -> M028/3(DW4)
  [in5] -> M028/4(P1W2)
  [in6] -> M028/5(P2W3)
  [in7] -> M028/6(P1W3)
  [in8] -> M028/7(P3W4)
  [in10] -> M028/8(O1)
  [in11] -> M028/9(O2)
  [in12] -> M028/10(O3)
  [in13] -> M028/11(O4)
  [in14] -> M028/12(LD)
  [in15] -> M028/13(CW1C)
  [in16] -> M028/14(CW2C)
  [in17] -> M028/15(CW3C)
  [in18] -> M028/16(CW4C)
  M028/1(W1Pos) -> Eval27/1(In1)
  M028/2(W2Pos) -> Eval27/2(In2)
  M028/3(W3Pos) -> Eval27/3(In3)
  M028/4(W4Pos) -> Eval27/4(In4)
  Eval27/1(Out1) -> To Workspace27/1
  [in1] -> M029/1(DW1)
  [in2] -> M029/2(DW2)
  [in4] -> M029/3(DW4)
  [in5] -> M029/4(P1W2)
  [in6] -> M029/5(P2W3)
  [in7] -> M029/6(P1W3)
  [in8] -> M029/7(P3W4)
  [in10] -> M029/8(O1)
  [in11] -> M029/9(O2)
  [in12] -> M029/10(O3)
  [in13] -> M029/11(O4)
  [in14] -> M029/12(LD)
  [in15] -> M029/13(CW1C)
  [in16] -> M029/14(CW2C)
  [in17] -> M029/15(CW3C)
  [in18] -> M029/16(CW4C)
  M029/1(W1Pos) -> Eval28/1(In1)
  M029/2(W2Pos) -> Eval28/2(In2)
  M029/3(W3Pos) -> Eval28/3(In3)
  M029/4(W4Pos) -> Eval28/4(In4)
  Eval28/1(Out1) -> To Workspace28/1
  [in1] -> M030/1(DW1)
  [in2] -> M030/2(DW2)
  [in4] -> M030/3(DW4)
  [in5] -> M030/4(P1W2)
  [in6] -> M030/5(P2W3)
  [in7] -> M030/6(P1W3)
  [in8] -> M030/7(P3W4)
  [in10] -> M030/8(O1)
  [in11] -> M030/9(O2)
  [in12] -> M030/10(O3)
  [in13] -> M030/11(O4)
  [in14] -> M030/12(LD)
  [in15] -> M030/13(CW1C)
  [in16] -> M030/14(CW2C)
  [in17] -> M030/15(CW3C)
  [in18] -> M030/16(CW4C)
  M030/1(W1Pos) -> Eval29/1(In1)
  M030/2(W2Pos) -> Eval29/2(In2)
  M030/3(W3Pos) -> Eval29/3(In3)
  M030/4(W4Pos) -> Eval29/4(In4)
  Eval29/1(Out1) -> To Workspace29/1
  [in1] -> M031/1(DW1)
  [in2] -> M031/2(DW2)
  [in4] -> M031/3(DW4)
  [in5] -> M031/4(P1W2)
  [in6] -> M031/5(P2W3)
  [in7] -> M031/6(P1W3)
  [in8] -> M031/7(P3W4)
  [in10] -> M031/8(O1)
  [in11] -> M031/9(O2)
  [in12] -> M031/10(O3)
  [in13] -> M031/11(O4)
  [in14] -> M031/12(LD)
  [in15] -> M031/13(CW1C)
  [in16] -> M031/14(CW2C)
  [in17] -> M031/15(CW3C)
  [in18] -> M031/16(CW4C)
  M031/1(W1Pos) -> Eval30/1(In1)
  M031/2(W2Pos) -> Eval30/2(In2)
  M031/3(W3Pos) -> Eval30/3(In3)
  M031/4(W4Pos) -> Eval30/4(In4)
  Eval30/1(Out1) -> To Workspace30/1
  [in1] -> M032/1(DW1)
  [in2] -> M032/2(DW2)
  [in4] -> M032/3(DW4)
  [in5] -> M032/4(P1W2)
  [in6] -> M032/5(P2W3)
  [in7] -> M032/6(P1W3)
  [in8] -> M032/7(P3W4)
  [in10] -> M032/8(O1)
  [in11] -> M032/9(O2)
  [in12] -> M032/10(O3)
  [in13] -> M032/11(O4)
  [in14] -> M032/12(LD)
  [in15] -> M032/13(CW1C)
  [in16] -> M032/14(CW2C)
  [in17] -> M032/15(CW3C)
  [in18] -> M032/16(CW4C)
  M032/1(W1Pos) -> Eval31/1(In1)
  M032/2(W2Pos) -> Eval31/2(In2)
  M032/3(W3Pos) -> Eval31/3(In3)
  M032/4(W4Pos) -> Eval31/4(In4)
  Eval31/1(Out1) -> To Workspace31/1
  [in1] -> M033/1(DW1)
  [in2] -> M033/2(DW2)
  [in4] -> M033/3(DW4)
  [in5] -> M033/4(P1W2)
  [in6] -> M033/5(P2W3)
  [in7] -> M033/6(P1W3)
  [in8] -> M033/7(P3W4)
  [in10] -> M033/8(O1)
  [in11] -> M033/9(O2)
  [in12] -> M033/10(O3)
  [in13] -> M033/11(O4)
  [in14] -> M033/12(LD)
  [in15] -> M033/13(CW1C)
  [in16] -> M033/14(CW2C)
  [in17] -> M033/15(CW3C)
  [in18] -> M033/16(CW4C)
  M033/1(W1Pos) -> Eval32/1(In1)
  M033/2(W2Pos) -> Eval32/2(In2)
  M033/3(W3Pos) -> Eval32/3(In3)
  M033/4(W4Pos) -> Eval32/4(In4)
  Eval32/1(Out1) -> To Workspace32/1
  [in1] -> M034/1(DW1)
  [in2] -> M034/2(DW2)
  [in4] -> M034/3(DW4)
  [in5] -> M034/4(P1W2)
  [in6] -> M034/5(P2W3)
  [in7] -> M034/6(P1W3)
  [in8] -> M034/7(P3W4)
  [in10] -> M034/8(O1)
  [in11] -> M034/9(O2)
  [in12] -> M034/10(O3)
  [in13] -> M034/11(O4)
  [in14] -> M034/12(LD)
  [in15] -> M034/13(CW1C)
  [in16] -> M034/14(CW2C)
  [in17] -> M034/15(CW3C)
  [in18] -> M034/16(CW4C)
  M034/1(W1Pos) -> Eval33/1(In1)
  M034/2(W2Pos) -> Eval33/2(In2)
  M034/3(W3Pos) -> Eval33/3(In3)
  M034/4(W4Pos) -> Eval33/4(In4)
  Eval33/1(Out1) -> To Workspace33/1
  [in1] -> M035/1(DW1)
  [in2] -> M035/2(DW2)
  [in4] -> M035/3(DW4)
  [in5] -> M035/4(P1W2)
  [in6] -> M035/5(P2W3)
  [in7] -> M035/6(P1W3)
  [in8] -> M035/7(P3W4)
  [in10] -> M035/8(O1)
  [in11] -> M035/9(O2)
  [in12] -> M035/10(O3)
  [in13] -> M035/11(O4)
  [in14] -> M035/12(LD)
  [in15] -> M035/13(CW1C)
  [in16] -> M035/14(CW2C)
  [in17] -> M035/15(CW3C)
  [in18] -> M035/16(CW4C)
  M035/1(W1Pos) -> Eval34/1(In1)
  M035/2(W2Pos) -> Eval34/2(In2)
  M035/3(W3Pos) -> Eval34/3(In3)
  M035/4(W4Pos) -> Eval34/4(In4)
  Eval34/1(Out1) -> To Workspace34/1
  [in1] -> M036/1(DW1)
  [in2] -> M036/2(DW2)
  [in4] -> M036/3(DW4)
  [in5] -> M036/4(P1W2)
  [in6] -> M036/5(P2W3)
  [in7] -> M036/6(P1W3)
  [in8] -> M036/7(P3W4)
  [in10] -> M036/8(O1)
  [in11] -> M036/9(O2)
  [in12] -> M036/10(O3)
  [in13] -> M036/11(O4)
  [in14] -> M036/12(LD)
  [in15] -> M036/13(CW1C)
  [in16] -> M036/14(CW2C)
  [in17] -> M036/15(CW3C)
  [in18] -> M036/16(CW4C)
  M036/1(W1Pos) -> Eval35/1(In1)
  M036/2(W2Pos) -> Eval35/2(In2)
  M036/3(W3Pos) -> Eval35/3(In3)
  M036/4(W4Pos) -> Eval35/4(In4)
  Eval35/1(Out1) -> To Workspace35/1
  [in1] -> M037/1(DW1)
  [in2] -> M037/2(DW2)
  [in4] -> M037/3(DW4)
  [in5] -> M037/4(P1W2)
  [in6] -> M037/5(P2W3)
  [in7] -> M037/6(P1W3)
  [in8] -> M037/7(P3W4)
  [in10] -> M037/8(O1)
  [in11] -> M037/9(O2)
  [in12] -> M037/10(O3)
  [in13] -> M037/11(O4)
  [in14] -> M037/12(LD)
  [in15] -> M037/13(CW1C)
  [in16] -> M037/14(CW2C)
  [in17] -> M037/15(CW3C)
  [in18] -> M037/16(CW4C)
  M037/1(W1Pos) -> Eval36/1(In1)
  M037/2(W2Pos) -> Eval36/2(In2)
  M037/3(W3Pos) -> Eval36/3(In3)
  M037/4(W4Pos) -> Eval36/4(In4)
  Eval36/1(Out1) -> To Workspace36/1
  [in1] -> M038/1(DW1)
  [in2] -> M038/2(DW2)
  [in4] -> M038/3(DW4)
  [in5] -> M038/4(P1W2)
  [in6] -> M038/5(P2W3)
  [in7] -> M038/6(P1W3)
  [in8] -> M038/7(P3W4)
  [in10] -> M038/8(O1)
  [in11] -> M038/9(O2)
  [in12] -> M038/10(O3)
  [in13] -> M038/11(O4)
  [in14] -> M038/12(LD)
  [in15] -> M038/13(CW1C)
  [in16] -> M038/14(CW2C)
  [in17] -> M038/15(CW3C)
  [in18] -> M038/16(CW4C)
  M038/1(W1Pos) -> Eval37/1(In1)
  M038/2(W2Pos) -> Eval37/2(In2)
  M038/3(W3Pos) -> Eval37/3(In3)
  M038/4(W4Pos) -> Eval37/4(In4)
  Eval37/1(Out1) -> To Workspace37/1
  [in1] -> M039/1(DW1)
  [in2] -> M039/2(DW2)
  [in4] -> M039/3(DW4)
  [in5] -> M039/4(P1W2)
  [in6] -> M039/5(P2W3)
  [in7] -> M039/6(P1W3)
  [in8] -> M039/7(P3W4)
  [in10] -> M039/8(O1)
  [in11] -> M039/9(O2)
  [in12] -> M039/10(O3)
  [in13] -> M039/11(O4)
  [in14] -> M039/12(LD)
  [in15] -> M039/13(CW1C)
  [in16] -> M039/14(CW2C)
  [in17] -> M039/15(CW3C)
  [in18] -> M039/16(CW4C)
  M039/1(W1Pos) -> Eval38/1(In1)
  M039/2(W2Pos) -> Eval38/2(In2)
  M039/3(W3Pos) -> Eval38/3(In3)
  M039/4(W4Pos) -> Eval38/4(In4)
  Eval38/1(Out1) -> To Workspace38/1
  [in1] -> M040/1(DW1)
  [in2] -> M040/2(DW2)
  [in4] -> M040/3(DW4)
  [in5] -> M040/4(P1W2)
  [in6] -> M040/5(P2W3)
  [in7] -> M040/6(P1W3)
  [in8] -> M040/7(P3W4)
  [in10] -> M040/8(O1)
  [in11] -> M040/9(O2)
  [in12] -> M040/10(O3)
  [in13] -> M040/11(O4)
  [in14] -> M040/12(LD)
  [in15] -> M040/13(CW1C)
  [in16] -> M040/14(CW2C)
  [in17] -> M040/15(CW3C)
  [in18] -> M040/16(CW4C)
  M040/1(W1Pos) -> Eval39/1(In1)
  M040/2(W2Pos) -> Eval39/2(In2)
  M040/3(W3Pos) -> Eval39/3(In3)
  M040/4(W4Pos) -> Eval39/4(In4)
  Eval39/1(Out1) -> To Workspace39/1
  [in1] -> M041/1(DW1)
  [in2] -> M041/2(DW2)
  [in4] -> M041/3(DW4)
  [in5] -> M041/4(P1W2)
  [in6] -> M041/5(P2W3)
  [in7] -> M041/6(P1W3)
  [in8] -> M041/7(P3W4)
  [in10] -> M041/8(O1)
  [in11] -> M041/9(O2)
  [in12] -> M041/10(O3)
  [in13] -> M041/11(O4)
  [in14] -> M041/12(LD)
  [in15] -> M041/13(CW1C)
  [in16] -> M041/14(CW2C)
  [in17] -> M041/15(CW3C)
  [in18] -> M041/16(CW4C)
  M041/1(W1Pos) -> Eval40/1(In1)
  M041/2(W2Pos) -> Eval40/2(In2)
  M041/3(W3Pos) -> Eval40/3(In3)
  M041/4(W4Pos) -> Eval40/4(In4)
  Eval40/1(Out1) -> To Workspace40/1
  [in1] -> M042/1(DW1)
  [in2] -> M042/2(DW2)
  [in4] -> M042/3(DW4)
  [in5] -> M042/4(P1W2)
  [in6] -> M042/5(P2W3)
  [in7] -> M042/6(P1W3)
  [in8] -> M042/7(P3W4)
  [in10] -> M042/8(O1)
  [in11] -> M042/9(O2)
  [in12] -> M042/10(O3)
  [in13] -> M042/11(O4)
  [in14] -> M042/12(LD)
  [in15] -> M042/13(CW1C)
  [in16] -> M042/14(CW2C)
  [in17] -> M042/15(CW3C)
  [in18] -> M042/16(CW4C)
  M042/1(W1Pos) -> Eval41/1(In1)
  M042/2(W2Pos) -> Eval41/2(In2)
  M042/3(W3Pos) -> Eval41/3(In3)
  M042/4(W4Pos) -> Eval41/4(In4)
  Eval41/1(Out1) -> To Workspace41/1
  [in1] -> M043/1(DW1)
  [in2] -> M043/2(DW2)
  [in4] -> M043/3(DW4)
  [in5] -> M043/4(P1W2)
  [in6] -> M043/5(P2W3)
  [in7] -> M043/6(P1W3)
  [in8] -> M043/7(P3W4)
  [in10] -> M043/8(O1)
  [in11] -> M043/9(O2)
  [in12] -> M043/10(O3)
  [in13] -> M043/11(O4)
  [in14] -> M043/12(LD)
  [in15] -> M043/13(CW1C)
  [in16] -> M043/14(CW2C)
  [in17] -> M043/15(CW3C)
  [in18] -> M043/16(CW4C)
  M043/1(W1Pos) -> Eval42/1(In1)
  M043/2(W2Pos) -> Eval42/2(In2)
  M043/3(W3Pos) -> Eval42/3(In3)
  M043/4(W4Pos) -> Eval42/4(In4)
  Eval42/1(Out1) -> To Workspace42/1
  [in1] -> M044/1(DW1)
  [in2] -> M044/2(DW2)
  [in4] -> M044/3(DW4)
  [in5] -> M044/4(P1W2)
  [in6] -> M044/5(P2W3)
  [in7] -> M044/6(P1W3)
  [in8] -> M044/7(P3W4)
  [in10] -> M044/8(O1)
  [in11] -> M044/9(O2)
  [in12] -> M044/10(O3)
  [in13] -> M044/11(O4)
  [in14] -> M044/12(LD)
  [in15] -> M044/13(CW1C)
  [in16] -> M044/14(CW2C)
  [in17] -> M044/15(CW3C)
  [in18] -> M044/16(CW4C)
  M044/1(W1Pos) -> Eval43/1(In1)
  M044/2(W2Pos) -> Eval43/2(In2)
  M044/3(W3Pos) -> Eval43/3(In3)
  M044/4(W4Pos) -> Eval43/4(In4)
  Eval43/1(Out1) -> To Workspace43/1
  [in1] -> M045/1(DW1)
  [in2] -> M045/2(DW2)
  [in4] -> M045/3(DW4)
  [in5] -> M045/4(P1W2)
  [in6] -> M045/5(P2W3)
  [in7] -> M045/6(P1W3)
  [in8] -> M045/7(P3W4)
  [in10] -> M045/8(O1)
  [in11] -> M045/9(O2)
  [in12] -> M045/10(O3)
  [in13] -> M045/11(O4)
  [in14] -> M045/12(LD)
  [in15] -> M045/13(CW1C)
  [in16] -> M045/14(CW2C)
  [in17] -> M045/15(CW3C)
  [in18] -> M045/16(CW4C)
  M045/1(W1Pos) -> Eval44/1(In1)
  M045/2(W2Pos) -> Eval44/2(In2)
  M045/3(W3Pos) -> Eval44/3(In3)
  M045/4(W4Pos) -> Eval44/4(In4)
  Eval44/1(Out1) -> To Workspace44/1
  [in1] -> M046/1(DW1)
  [in2] -> M046/2(DW2)
  [in4] -> M046/3(DW4)
  [in5] -> M046/4(P1W2)
  [in6] -> M046/5(P2W3)
  [in7] -> M046/6(P1W3)
  [in8] -> M046/7(P3W4)
  [in10] -> M046/8(O1)
  [in11] -> M046/9(O2)
  [in12] -> M046/10(O3)
  [in13] -> M046/11(O4)
  [in14] -> M046/12(LD)
  [in15] -> M046/13(CW1C)
  [in16] -> M046/14(CW2C)
  [in17] -> M046/15(CW3C)
  [in18] -> M046/16(CW4C)
  M046/1(W1Pos) -> Eval45/1(In1)
  M046/2(W2Pos) -> Eval45/2(In2)
  M046/3(W3Pos) -> Eval45/3(In3)
  M046/4(W4Pos) -> Eval45/4(In4)
  Eval45/1(Out1) -> To Workspace45/1
  [in1] -> M047/1(DW1)
  [in2] -> M047/2(DW2)
  [in4] -> M047/3(DW4)
  [in5] -> M047/4(P1W2)
  [in6] -> M047/5(P2W3)
  [in7] -> M047/6(P1W3)
  [in8] -> M047/7(P3W4)
  [in10] -> M047/8(O1)
  [in11] -> M047/9(O2)
  [in12] -> M047/10(O3)
  [in13] -> M047/11(O4)
  [in14] -> M047/12(LD)
  [in15] -> M047/13(CW1C)
  [in16] -> M047/14(CW2C)
  [in17] -> M047/15(CW3C)
  [in18] -> M047/16(CW4C)
  M047/1(W1Pos) -> Eval46/1(In1)
  M047/2(W2Pos) -> Eval46/2(In2)
  M047/3(W3Pos) -> Eval46/3(In3)
  M047/4(W4Pos) -> Eval46/4(In4)
  Eval46/1(Out1) -> To Workspace46/1
  [in1] -> M048/1(DW1)
  [in2] -> M048/2(DW2)
  [in4] -> M048/3(DW4)
  [in5] -> M048/4(P1W2)
  [in6] -> M048/5(P2W3)
  [in7] -> M048/6(P1W3)
  [in8] -> M048/7(P3W4)
  [in10] -> M048/8(O1)
  [in11] -> M048/9(O2)
  [in12] -> M048/10(O3)
  [in13] -> M048/11(O4)
  [in14] -> M048/12(LD)
  [in15] -> M048/13(CW1C)
  [in16] -> M048/14(CW2C)
  [in17] -> M048/15(CW3C)
  [in18] -> M048/16(CW4C)
  M048/1(W1Pos) -> Eval47/1(In1)
  M048/2(W2Pos) -> Eval47/2(In2)
  M048/3(W3Pos) -> Eval47/3(In3)
  M048/4(W4Pos) -> Eval47/4(In4)
  Eval47/1(Out1) -> To Workspace47/1
  [in1] -> M049/1(DW1)
  [in2] -> M049/2(DW2)
  [in4] -> M049/3(DW4)
  [in5] -> M049/4(P1W2)
  [in6] -> M049/5(P2W3)
  [in7] -> M049/6(P1W3)
  [in8] -> M049/7(P3W4)
  [in10] -> M049/8(O1)
  [in11] -> M049/9(O2)
  [in12] -> M049/10(O3)
  [in13] -> M049/11(O4)
  [in14] -> M049/12(LD)
  [in15] -> M049/13(CW1C)
  [in16] -> M049/14(CW2C)
  [in17] -> M049/15(CW3C)
  [in18] -> M049/16(CW4C)
  M049/1(W1Pos) -> Eval48/1(In1)
  M049/2(W2Pos) -> Eval48/2(In2)
  M049/3(W3Pos) -> Eval48/3(In3)
  M049/4(W4Pos) -> Eval48/4(In4)
  Eval48/1(Out1) -> To Workspace48/1
  [in1] -> M050/1(DW1)
  [in2] -> M050/2(DW2)
  [in4] -> M050/3(DW4)
  [in5] -> M050/4(P1W2)
  [in6] -> M050/5(P2W3)
  [in7] -> M050/6(P1W3)
  [in8] -> M050/7(P3W4)
  [in10] -> M050/8(O1)
  [in11] -> M050/9(O2)
  [in12] -> M050/10(O3)
  [in13] -> M050/11(O4)
  [in14] -> M050/12(LD)
  [in15] -> M050/13(CW1C)
  [in16] -> M050/14(CW2C)
  [in17] -> M050/15(CW3C)
  [in18] -> M050/16(CW4C)
  M050/1(W1Pos) -> Eval49/1(In1)
  M050/2(W2Pos) -> Eval49/2(In2)
  M050/3(W3Pos) -> Eval49/3(In3)
  M050/4(W4Pos) -> Eval49/4(In4)
  Eval49/1(Out1) -> To Workspace49/1
  [in1] -> M051/1(DW1)
  [in2] -> M051/2(DW2)
  [in4] -> M051/3(DW4)
  [in5] -> M051/4(P1W2)
  [in6] -> M051/5(P2W3)
  [in7] -> M051/6(P1W3)
  [in8] -> M051/7(P3W4)
  [in10] -> M051/8(O1)
  [in11] -> M051/9(O2)
  [in12] -> M051/10(O3)
  [in13] -> M051/11(O4)
  [in14] -> M051/12(LD)
  [in15] -> M051/13(CW1C)
  [in16] -> M051/14(CW2C)
  [in17] -> M051/15(CW3C)
  [in18] -> M051/16(CW4C)
  M051/1(W1Pos) -> Eval50/1(In1)
  M051/2(W2Pos) -> Eval50/2(In2)
  M051/3(W3Pos) -> Eval50/3(In3)
  M051/4(W4Pos) -> Eval50/4(In4)
  Eval50/1(Out1) -> To Workspace50/1
  [in1] -> M052/1(DW1)
  [in2] -> M052/2(DW2)
  [in4] -> M052/3(DW4)
  [in5] -> M052/4(P1W2)
  [in6] -> M052/5(P2W3)
  [in7] -> M052/6(P1W3)
  [in8] -> M052/7(P3W4)
  [in10] -> M052/8(O1)
  [in11] -> M052/9(O2)
  [in12] -> M052/10(O3)
  [in13] -> M052/11(O4)
  [in14] -> M052/12(LD)
  [in15] -> M052/13(CW1C)
  [in16] -> M052/14(CW2C)
  [in17] -> M052/15(CW3C)
  [in18] -> M052/16(CW4C)
  M052/1(W1Pos) -> Eval51/1(In1)
  M052/2(W2Pos) -> Eval51/2(In2)
  M052/3(W3Pos) -> Eval51/3(In3)
  M052/4(W4Pos) -> Eval51/4(In4)
  Eval51/1(Out1) -> To Workspace51/1
  [in1] -> M053/1(DW1)
  [in2] -> M053/2(DW2)
  [in4] -> M053/3(DW4)
  [in5] -> M053/4(P1W2)
  [in6] -> M053/5(P2W3)
  [in7] -> M053/6(P1W3)
  [in8] -> M053/7(P3W4)
  [in10] -> M053/8(O1)
  [in11] -> M053/9(O2)
  [in12] -> M053/10(O3)
  [in13] -> M053/11(O4)
  [in14] -> M053/12(LD)
  [in15] -> M053/13(CW1C)
  [in16] -> M053/14(CW2C)
  [in17] -> M053/15(CW3C)
  [in18] -> M053/16(CW4C)
  M053/1(W1Pos) -> Eval52/1(In1)
  M053/2(W2Pos) -> Eval52/2(In2)
  M053/3(W3Pos) -> Eval52/3(In3)
  M053/4(W4Pos) -> Eval52/4(In4)
  Eval52/1(Out1) -> To Workspace52/1
  [in1] -> M054/1(DW1)
  [in2] -> M054/2(DW2)
  [in4] -> M054/3(DW4)
  [in5] -> M054/4(P1W2)
  [in6] -> M054/5(P2W3)
  [in7] -> M054/6(P1W3)
  [in8] -> M054/7(P3W4)
  [in10] -> M054/8(O1)
  [in11] -> M054/9(O2)
  [in12] -> M054/10(O3)
  [in13] -> M054/11(O4)
  [in14] -> M054/12(LD)
  [in15] -> M054/13(CW1C)
  [in16] -> M054/14(CW2C)
  [in17] -> M054/15(CW3C)
  [in18] -> M054/16(CW4C)
  M054/1(W1Pos) -> Eval53/1(In1)
  M054/2(W2Pos) -> Eval53/2(In2)
  M054/3(W3Pos) -> Eval53/3(In3)
  M054/4(W4Pos) -> Eval53/4(In4)
  Eval53/1(Out1) -> To Workspace53/1
  [in1] -> M055/1(DW1)
  [in2] -> M055/2(DW2)
  [in4] -> M055/3(DW4)
  [in5] -> M055/4(P1W2)
  [in6] -> M055/5(P2W3)
  [in7] -> M055/6(P1W3)
  [in8] -> M055/7(P3W4)
  [in10] -> M055/8(O1)
  [in11] -> M055/9(O2)
  [in12] -> M055/10(O3)
  [in13] -> M055/11(O4)
  [in14] -> M055/12(LD)
  [in15] -> M055/13(CW1C)
  [in16] -> M055/14(CW2C)
  [in17] -> M055/15(CW3C)
  [in18] -> M055/16(CW4C)
  M055/1(W1Pos) -> Eval54/1(In1)
  M055/2(W2Pos) -> Eval54/2(In2)
  M055/3(W3Pos) -> Eval54/3(In3)
  M055/4(W4Pos) -> Eval54/4(In4)
  Eval54/1(Out1) -> To Workspace54/1
  [in1] -> M056/1(DW1)
  [in2] -> M056/2(DW2)
  [in4] -> M056/3(DW4)
  [in5] -> M056/4(P1W2)
  [in6] -> M056/5(P2W3)
  [in7] -> M056/6(P1W3)
  [in8] -> M056/7(P3W4)
  [in10] -> M056/8(O1)
  [in11] -> M056/9(O2)
  [in12] -> M056/10(O3)
  [in13] -> M056/11(O4)
  [in14] -> M056/12(LD)
  [in15] -> M056/13(CW1C)
  [in16] -> M056/14(CW2C)
  [in17] -> M056/15(CW3C)
  [in18] -> M056/16(CW4C)
  M056/1(W1Pos) -> Eval55/1(In1)
  M056/2(W2Pos) -> Eval55/2(In2)
  M056/3(W3Pos) -> Eval55/3(In3)
  M056/4(W4Pos) -> Eval55/4(In4)
  Eval55/1(Out1) -> To Workspace55/1
  [in1] -> M057/1(DW1)
  [in2] -> M057/2(DW2)
  [in4] -> M057/3(DW4)
  [in5] -> M057/4(P1W2)
  [in6] -> M057/5(P2W3)
  [in7] -> M057/6(P1W3)
  [in8] -> M057/7(P3W4)
  [in10] -> M057/8(O1)
  [in11] -> M057/9(O2)
  [in12] -> M057/10(O3)
  [in13] -> M057/11(O4)
  [in14] -> M057/12(LD)
  [in15] -> M057/13(CW1C)
  [in16] -> M057/14(CW2C)
  [in17] -> M057/15(CW3C)
  [in18] -> M057/16(CW4C)
  M057/1(W1Pos) -> Eval56/1(In1)
  M057/2(W2Pos) -> Eval56/2(In2)
  M057/3(W3Pos) -> Eval56/3(In3)
  M057/4(W4Pos) -> Eval56/4(In4)
  Eval56/1(Out1) -> To Workspace56/1
  [in1] -> M058/1(DW1)
  [in2] -> M058/2(DW2)
  [in4] -> M058/3(DW4)
  [in5] -> M058/4(P1W2)
  [in6] -> M058/5(P2W3)
  [in7] -> M058/6(P1W3)
  [in8] -> M058/7(P3W4)
  [in10] -> M058/8(O1)
  [in11] -> M058/9(O2)
  [in12] -> M058/10(O3)
  [in13] -> M058/11(O4)
  [in14] -> M058/12(LD)
  [in15] -> M058/13(CW1C)
  [in16] -> M058/14(CW2C)
  [in17] -> M058/15(CW3C)
  [in18] -> M058/16(CW4C)
  M058/1(W1Pos) -> Eval57/1(In1)
  M058/2(W2Pos) -> Eval57/2(In2)
  M058/3(W3Pos) -> Eval57/3(In3)
  M058/4(W4Pos) -> Eval57/4(In4)
  Eval57/1(Out1) -> To Workspace57/1
  [in1] -> M059/1(DW1)
  [in2] -> M059/2(DW2)
  [in4] -> M059/3(DW4)
  [in5] -> M059/4(P1W2)
  [in6] -> M059/5(P2W3)
  [in7] -> M059/6(P1W3)
  [in8] -> M059/7(P3W4)
  [in10] -> M059/8(O1)
  [in11] -> M059/9(O2)
  [in12] -> M059/10(O3)
  [in13] -> M059/11(O4)
  [in14] -> M059/12(LD)
  [in15] -> M059/13(CW1C)
  [in16] -> M059/14(CW2C)
  [in17] -> M059/15(CW3C)
  [in18] -> M059/16(CW4C)
  M059/1(W1Pos) -> Eval58/1(In1)
  M059/2(W2Pos) -> Eval58/2(In2)
  M059/3(W3Pos) -> Eval58/3(In3)
  M059/4(W4Pos) -> Eval58/4(In4)
  Eval58/1(Out1) -> To Workspace58/1
  [in1] -> M060/1(DW1)
  [in2] -> M060/2(DW2)
  [in4] -> M060/3(DW4)
  [in5] -> M060/4(P1W2)
  [in6] -> M060/5(P2W3)
  [in7] -> M060/6(P1W3)
  [in8] -> M060/7(P3W4)
  [in10] -> M060/8(O1)
  [in11] -> M060/9(O2)
  [in12] -> M060/10(O3)
  [in13] -> M060/11(O4)
  [in14] -> M060/12(LD)
  [in15] -> M060/13(CW1C)
  [in16] -> M060/14(CW2C)
  [in17] -> M060/15(CW3C)
  [in18] -> M060/16(CW4C)
  M060/1(W1Pos) -> Eval59/1(In1)
  M060/2(W2Pos) -> Eval59/2(In2)
  M060/3(W3Pos) -> Eval59/3(In3)
  M060/4(W4Pos) -> Eval59/4(In4)
  Eval59/1(Out1) -> To Workspace59/1
  [in1] -> M061/1(DW1)
  [in2] -> M061/2(DW2)
  [in4] -> M061/3(DW4)
  [in5] -> M061/4(P1W2)
  [in6] -> M061/5(P2W3)
  [in7] -> M061/6(P1W3)
  [in8] -> M061/7(P3W4)
  [in10] -> M061/8(O1)
  [in11] -> M061/9(O2)
  [in12] -> M061/10(O3)
  [in13] -> M061/11(O4)
  [in14] -> M061/12(LD)
  [in15] -> M061/13(CW1C)
  [in16] -> M061/14(CW2C)
  [in17] -> M061/15(CW3C)
  [in18] -> M061/16(CW4C)
  M061/1(W1Pos) -> Eval60/1(In1)
  M061/2(W2Pos) -> Eval60/2(In2)
  M061/3(W3Pos) -> Eval60/3(In3)
  M061/4(W4Pos) -> Eval60/4(In4)
  Eval60/1(Out1) -> To Workspace60/1
  [in1] -> M062/1(DW1)
  [in2] -> M062/2(DW2)
  [in4] -> M062/3(DW4)
  [in5] -> M062/4(P1W2)
  [in6] -> M062/5(P2W3)
  [in7] -> M062/6(P1W3)
  [in8] -> M062/7(P3W4)
  [in10] -> M062/8(O1)
  [in11] -> M062/9(O2)
  [in12] -> M062/10(O3)
  [in13] -> M062/11(O4)
  [in14] -> M062/12(LD)
  [in15] -> M062/13(CW1C)
  [in16] -> M062/14(CW2C)
  [in17] -> M062/15(CW3C)
  [in18] -> M062/16(CW4C)
  M062/1(W1Pos) -> Eval61/1(In1)
  M062/2(W2Pos) -> Eval61/2(In2)
  M062/3(W3Pos) -> Eval61/3(In3)
  M062/4(W4Pos) -> Eval61/4(In4)
  Eval61/1(Out1) -> To Workspace61/1
  [in1] -> M063/1(DW1)
  [in2] -> M063/2(DW2)
  [in4] -> M063/3(DW4)
  [in5] -> M063/4(P1W2)
  [in6] -> M063/5(P2W3)
  [in7] -> M063/6(P1W3)
  [in8] -> M063/7(P3W4)
  [in10] -> M063/8(O1)
  [in11] -> M063/9(O2)
  [in12] -> M063/10(O3)
  [in13] -> M063/11(O4)
  [in14] -> M063/12(LD)
  [in15] -> M063/13(CW1C)
  [in16] -> M063/14(CW2C)
  [in17] -> M063/15(CW3C)
  [in18] -> M063/16(CW4C)
  M063/1(W1Pos) -> Eval62/1(In1)
  M063/2(W2Pos) -> Eval62/2(In2)
  M063/3(W3Pos) -> Eval62/3(In3)
  M063/4(W4Pos) -> Eval62/4(In4)
  Eval62/1(Out1) -> To Workspace62/1
  [in1] -> M064/1(DW1)
  [in2] -> M064/2(DW2)
  [in4] -> M064/3(DW4)
  [in5] -> M064/4(P1W2)
  [in6] -> M064/5(P2W3)
  [in7] -> M064/6(P1W3)
  [in8] -> M064/7(P3W4)
  [in10] -> M064/8(O1)
  [in11] -> M064/9(O2)
  [in12] -> M064/10(O3)
  [in13] -> M064/11(O4)
  [in14] -> M064/12(LD)
  [in15] -> M064/13(CW1C)
  [in16] -> M064/14(CW2C)
  [in17] -> M064/15(CW3C)
  [in18] -> M064/16(CW4C)
  M064/1(W1Pos) -> Eval63/1(In1)
  M064/2(W2Pos) -> Eval63/2(In2)
  M064/3(W3Pos) -> Eval63/3(In3)
  M064/4(W4Pos) -> Eval63/4(In4)
  Eval63/1(Out1) -> To Workspace63/1
  [in1] -> M065/1(DW1)
  [in2] -> M065/2(DW2)
  [in4] -> M065/3(DW4)
  [in5] -> M065/4(P1W2)
  [in6] -> M065/5(P2W3)
  [in7] -> M065/6(P1W3)
  [in8] -> M065/7(P3W4)
  [in10] -> M065/8(O1)
  [in11] -> M065/9(O2)
  [in12] -> M065/10(O3)
  [in13] -> M065/11(O4)
  [in14] -> M065/12(LD)
  [in15] -> M065/13(CW1C)
  [in16] -> M065/14(CW2C)
  [in17] -> M065/15(CW3C)
  [in18] -> M065/16(CW4C)
  M065/1(W1Pos) -> Eval64/1(In1)
  M065/2(W2Pos) -> Eval64/2(In2)
  M065/3(W3Pos) -> Eval64/3(In3)
  M065/4(W4Pos) -> Eval64/4(In4)
  Eval64/1(Out1) -> To Workspace64/1
  [in1] -> M066/1(DW1)
  [in2] -> M066/2(DW2)
  [in4] -> M066/3(DW4)
  [in5] -> M066/4(P1W2)
  [in6] -> M066/5(P2W3)
  [in7] -> M066/6(P1W3)
  [in8] -> M066/7(P3W4)
  [in10] -> M066/8(O1)
  [in11] -> M066/9(O2)
  [in12] -> M066/10(O3)
  [in13] -> M066/11(O4)
  [in14] -> M066/12(LD)
  [in15] -> M066/13(CW1C)
  [in16] -> M066/14(CW2C)
  [in17] -> M066/15(CW3C)
  [in18] -> M066/16(CW4C)
  M066/1(W1Pos) -> Eval65/1(In1)
  M066/2(W2Pos) -> Eval65/2(In2)
  M066/3(W3Pos) -> Eval65/3(In3)
  M066/4(W4Pos) -> Eval65/4(In4)
  Eval65/1(Out1) -> To Workspace65/1
  [in1] -> M067/1(DW1)
  [in2] -> M067/2(DW2)
  [in4] -> M067/3(DW4)
  [in5] -> M067/4(P1W2)
  [in6] -> M067/5(P2W3)
  [in7] -> M067/6(P1W3)
  [in8] -> M067/7(P3W4)
  [in10] -> M067/8(O1)
  [in11] -> M067/9(O2)
  [in12] -> M067/10(O3)
  [in13] -> M067/11(O4)
  [in14] -> M067/12(LD)
  [in15] -> M067/13(CW1C)
  [in16] -> M067/14(CW2C)
  [in17] -> M067/15(CW3C)
  [in18] -> M067/16(CW4C)
  M067/1(W1Pos) -> Eval66/1(In1)
  M067/2(W2Pos) -> Eval66/2(In2)
  M067/3(W3Pos) -> Eval66/3(In3)
  M067/4(W4Pos) -> Eval66/4(In4)
  Eval66/1(Out1) -> To Workspace66/1
  [in1] -> M068/1(DW1)
  [in2] -> M068/2(DW2)
  [in4] -> M068/3(DW4)
  [in5] -> M068/4(P1W2)
  [in6] -> M068/5(P2W3)
  [in7] -> M068/6(P1W3)
  [in8] -> M068/7(P3W4)
  [in10] -> M068/8(O1)
  [in11] -> M068/9(O2)
  [in12] -> M068/10(O3)
  [in13] -> M068/11(O4)
  [in14] -> M068/12(LD)
  [in15] -> M068/13(CW1C)
  [in16] -> M068/14(CW2C)
  [in17] -> M068/15(CW3C)
  [in18] -> M068/16(CW4C)
  M068/1(W1Pos) -> Eval67/1(In1)
  M068/2(W2Pos) -> Eval67/2(In2)
  M068/3(W3Pos) -> Eval67/3(In3)
  M068/4(W4Pos) -> Eval67/4(In4)
  Eval67/1(Out1) -> To Workspace67/1
  [in1] -> M069/1(DW1)
  [in2] -> M069/2(DW2)
  [in4] -> M069/3(DW4)
  [in5] -> M069/4(P1W2)
  [in6] -> M069/5(P2W3)
  [in7] -> M069/6(P1W3)
  [in8] -> M069/7(P3W4)
  [in10] -> M069/8(O1)
  [in11] -> M069/9(O2)
  [in12] -> M069/10(O3)
  [in13] -> M069/11(O4)
  [in14] -> M069/12(LD)
  [in15] -> M069/13(CW1C)
  [in16] -> M069/14(CW2C)
  [in17] -> M069/15(CW3C)
  [in18] -> M069/16(CW4C)
  M069/1(W1Pos) -> Eval68/1(In1)
  M069/2(W2Pos) -> Eval68/2(In2)
  M069/3(W3Pos) -> Eval68/3(In3)
  M069/4(W4Pos) -> Eval68/4(In4)
  Eval68/1(Out1) -> To Workspace68/1
  [in1] -> M070/1(DW1)
  [in2] -> M070/2(DW2)
  [in4] -> M070/3(DW4)
  [in5] -> M070/4(P1W2)
  [in6] -> M070/5(P2W3)
  [in7] -> M070/6(P1W3)
  [in8] -> M070/7(P3W4)
  [in10] -> M070/8(O1)
  [in11] -> M070/9(O2)
  [in12] -> M070/10(O3)
  [in13] -> M070/11(O4)
  [in14] -> M070/12(LD)
  [in15] -> M070/13(CW1C)
  [in16] -> M070/14(CW2C)
  [in17] -> M070/15(CW3C)
  [in18] -> M070/16(CW4C)
  M070/1(W1Pos) -> Eval69/1(In1)
  M070/2(W2Pos) -> Eval69/2(In2)
  M070/3(W3Pos) -> Eval69/3(In3)
  M070/4(W4Pos) -> Eval69/4(In4)
  Eval69/1(Out1) -> To Workspace69/1
  [in1] -> M071/1(DW1)
  [in2] -> M071/2(DW2)
  [in4] -> M071/3(DW4)
  [in5] -> M071/4(P1W2)
  [in6] -> M071/5(P2W3)
  [in7] -> M071/6(P1W3)
  [in8] -> M071/7(P3W4)
  [in10] -> M071/8(O1)
  [in11] -> M071/9(O2)
  [in12] -> M071/10(O3)
  [in13] -> M071/11(O4)
  [in14] -> M071/12(LD)
  [in15] -> M071/13(CW1C)
  [in16] -> M071/14(CW2C)
  [in17] -> M071/15(CW3C)
  [in18] -> M071/16(CW4C)
  M071/1(W1Pos) -> Eval70/1(In1)
  M071/2(W2Pos) -> Eval70/2(In2)
  M071/3(W3Pos) -> Eval70/3(In3)
  M071/4(W4Pos) -> Eval70/4(In4)
  Eval70/1(Out1) -> To Workspace70/1
  [in1] -> M072/1(DW1)
  [in2] -> M072/2(DW2)
  [in4] -> M072/3(DW4)
  [in5] -> M072/4(P1W2)
  [in6] -> M072/5(P2W3)
  [in7] -> M072/6(P1W3)
  [in8] -> M072/7(P3W4)
  [in10] -> M072/8(O1)
  [in11] -> M072/9(O2)
  [in12] -> M072/10(O3)
  [in13] -> M072/11(O4)
  [in14] -> M072/12(LD)
  [in15] -> M072/13(CW1C)
  [in16] -> M072/14(CW2C)
  [in17] -> M072/15(CW3C)
  [in18] -> M072/16(CW4C)
  M072/1(W1Pos) -> Eval71/1(In1)
  M072/2(W2Pos) -> Eval71/2(In2)
  M072/3(W3Pos) -> Eval71/3(In3)
  M072/4(W4Pos) -> Eval71/4(In4)
  Eval71/1(Out1) -> To Workspace71/1
  [in1] -> M073/1(DW1)
  [in2] -> M073/2(DW2)
  [in4] -> M073/3(DW4)
  [in5] -> M073/4(P1W2)
  [in6] -> M073/5(P2W3)
  [in7] -> M073/6(P1W3)
  [in8] -> M073/7(P3W4)
  [in10] -> M073/8(O1)
  [in11] -> M073/9(O2)
  [in12] -> M073/10(O3)
  [in13] -> M073/11(O4)
  [in14] -> M073/12(LD)
  [in15] -> M073/13(CW1C)
  [in16] -> M073/14(CW2C)
  [in17] -> M073/15(CW3C)
  [in18] -> M073/16(CW4C)
  M073/1(W1Pos) -> Eval72/1(In1)
  M073/2(W2Pos) -> Eval72/2(In2)
  M073/3(W3Pos) -> Eval72/3(In3)
  M073/4(W4Pos) -> Eval72/4(In4)
  Eval72/1(Out1) -> To Workspace72/1
  [in1] -> M074/1(DW1)
  [in2] -> M074/2(DW2)
  [in4] -> M074/3(DW4)
  [in5] -> M074/4(P1W2)
  [in6] -> M074/5(P2W3)
  [in7] -> M074/6(P1W3)
  [in8] -> M074/7(P3W4)
  [in10] -> M074/8(O1)
  [in11] -> M074/9(O2)
  [in12] -> M074/10(O3)
  [in13] -> M074/11(O4)
  [in14] -> M074/12(LD)
  [in15] -> M074/13(CW1C)
  [in16] -> M074/14(CW2C)
  [in17] -> M074/15(CW3C)
  [in18] -> M074/16(CW4C)
  M074/1(W1Pos) -> Eval73/1(In1)
  M074/2(W2Pos) -> Eval73/2(In2)
  M074/3(W3Pos) -> Eval73/3(In3)
  M074/4(W4Pos) -> Eval73/4(In4)
  Eval73/1(Out1) -> To Workspace73/1
  [in1] -> M075/1(DW1)
  [in2] -> M075/2(DW2)
  [in4] -> M075/3(DW4)
  [in5] -> M075/4(P1W2)
  [in6] -> M075/5(P2W3)
  [in7] -> M075/6(P1W3)
  [in8] -> M075/7(P3W4)
  [in10] -> M075/8(O1)
  [in11] -> M075/9(O2)
  [in12] -> M075/10(O3)
  [in13] -> M075/11(O4)
  [in14] -> M075/12(LD)
  [in15] -> M075/13(CW1C)
  [in16] -> M075/14(CW2C)
  [in17] -> M075/15(CW3C)
  [in18] -> M075/16(CW4C)
  M075/1(W1Pos) -> Eval74/1(In1)
  M075/2(W2Pos) -> Eval74/2(In2)
  M075/3(W3Pos) -> Eval74/3(In3)
  M075/4(W4Pos) -> Eval74/4(In4)
  Eval74/1(Out1) -> To Workspace74/1
  [in1] -> M076/1(DW1)
  [in2] -> M076/2(DW2)
  [in4] -> M076/3(DW4)
  [in5] -> M076/4(P1W2)
  [in6] -> M076/5(P2W3)
  [in7] -> M076/6(P1W3)
  [in8] -> M076/7(P3W4)
  [in10] -> M076/8(O1)
  [in11] -> M076/9(O2)
  [in12] -> M076/10(O3)
  [in13] -> M076/11(O4)
  [in14] -> M076/12(LD)
  [in15] -> M076/13(CW1C)
  [in16] -> M076/14(CW2C)
  [in17] -> M076/15(CW3C)
  [in18] -> M076/16(CW4C)
  M076/1(W1Pos) -> Eval75/1(In1)
  M076/2(W2Pos) -> Eval75/2(In2)
  M076/3(W3Pos) -> Eval75/3(In3)
  M076/4(W4Pos) -> Eval75/4(In4)
  Eval75/1(Out1) -> To Workspace75/1
  [in1] -> M077/1(DW1)
  [in2] -> M077/2(DW2)
  [in4] -> M077/3(DW4)
  [in5] -> M077/4(P1W2)
  [in6] -> M077/5(P2W3)
  [in7] -> M077/6(P1W3)
  [in8] -> M077/7(P3W4)
  [in10] -> M077/8(O1)
  [in11] -> M077/9(O2)
  [in12] -> M077/10(O3)
  [in13] -> M077/11(O4)
  [in14] -> M077/12(LD)
  [in15] -> M077/13(CW1C)
  [in16] -> M077/14(CW2C)
  [in17] -> M077/15(CW3C)
  [in18] -> M077/16(CW4C)
  M077/1(W1Pos) -> Eval76/1(In1)
  M077/2(W2Pos) -> Eval76/2(In2)
  M077/3(W3Pos) -> Eval76/3(In3)
  M077/4(W4Pos) -> Eval76/4(In4)
  Eval76/1(Out1) -> To Workspace76/1
  [in1] -> M078/1(DW1)
  [in2] -> M078/2(DW2)
  [in4] -> M078/3(DW4)
  [in5] -> M078/4(P1W2)
  [in6] -> M078/5(P2W3)
  [in7] -> M078/6(P1W3)
  [in8] -> M078/7(P3W4)
  [in10] -> M078/8(O1)
  [in11] -> M078/9(O2)
  [in12] -> M078/10(O3)
  [in13] -> M078/11(O4)
  [in14] -> M078/12(LD)
  [in15] -> M078/13(CW1C)
  [in16] -> M078/14(CW2C)
  [in17] -> M078/15(CW3C)
  [in18] -> M078/16(CW4C)
  M078/1(W1Pos) -> Eval77/1(In1)
  M078/2(W2Pos) -> Eval77/2(In2)
  M078/3(W3Pos) -> Eval77/3(In3)
  M078/4(W4Pos) -> Eval77/4(In4)
  Eval77/1(Out1) -> To Workspace77/1
  [in1] -> M079/1(DW1)
  [in2] -> M079/2(DW2)
  [in4] -> M079/3(DW4)
  [in5] -> M079/4(P1W2)
  [in6] -> M079/5(P2W3)
  [in7] -> M079/6(P1W3)
  [in8] -> M079/7(P3W4)
  [in10] -> M079/8(O1)
  [in11] -> M079/9(O2)
  [in12] -> M079/10(O3)
  [in13] -> M079/11(O4)
  [in14] -> M079/12(LD)
  [in15] -> M079/13(CW1C)
  [in16] -> M079/14(CW2C)
  [in17] -> M079/15(CW3C)
  [in18] -> M079/16(CW4C)
  M079/1(W1Pos) -> Eval78/1(In1)
  M079/2(W2Pos) -> Eval78/2(In2)
  M079/3(W3Pos) -> Eval78/3(In3)
  M079/4(W4Pos) -> Eval78/4(In4)
  Eval78/1(Out1) -> To Workspace78/1
  [in1] -> M080/1(DW1)
  [in2] -> M080/2(DW2)
  [in4] -> M080/3(DW4)
  [in5] -> M080/4(P1W2)
  [in6] -> M080/5(P2W3)
  [in7] -> M080/6(P1W3)
  [in8] -> M080/7(P3W4)
  [in10] -> M080/8(O1)
  [in11] -> M080/9(O2)
  [in12] -> M080/10(O3)
  [in13] -> M080/11(O4)
  [in14] -> M080/12(LD)
  [in15] -> M080/13(CW1C)
  [in16] -> M080/14(CW2C)
  [in17] -> M080/15(CW3C)
  [in18] -> M080/16(CW4C)
  M080/1(W1Pos) -> Eval79/1(In1)
  M080/2(W2Pos) -> Eval79/2(In2)
  M080/3(W3Pos) -> Eval79/3(In3)
  M080/4(W4Pos) -> Eval79/4(In4)
  Eval79/1(Out1) -> To Workspace79/1
  [in1] -> M081/1(DW1)
  [in2] -> M081/2(DW2)
  [in4] -> M081/3(DW4)
  [in5] -> M081/4(P1W2)
  [in6] -> M081/5(P2W3)
  [in7] -> M081/6(P1W3)
  [in8] -> M081/7(P3W4)
  [in10] -> M081/8(O1)
  [in11] -> M081/9(O2)
  [in12] -> M081/10(O3)
  [in13] -> M081/11(O4)
  [in14] -> M081/12(LD)
  [in15] -> M081/13(CW1C)
  [in16] -> M081/14(CW2C)
  [in17] -> M081/15(CW3C)
  [in18] -> M081/16(CW4C)
  M081/1(W1Pos) -> Eval80/1(In1)
  M081/2(W2Pos) -> Eval80/2(In2)
  M081/3(W3Pos) -> Eval80/3(In3)
  M081/4(W4Pos) -> Eval80/4(In4)
  Eval80/1(Out1) -> To Workspace80/1
  [in1] -> M082/1(DW1)
  [in2] -> M082/2(DW2)
  [in4] -> M082/3(DW4)
  [in5] -> M082/4(P1W2)
  [in6] -> M082/5(P2W3)
  [in7] -> M082/6(P1W3)
  [in8] -> M082/7(P3W4)
  [in10] -> M082/8(O1)
  [in11] -> M082/9(O2)
  [in12] -> M082/10(O3)
  [in13] -> M082/11(O4)
  [in14] -> M082/12(LD)
  [in15] -> M082/13(CW1C)
  [in16] -> M082/14(CW2C)
  [in17] -> M082/15(CW3C)
  [in18] -> M082/16(CW4C)
  M082/1(W1Pos) -> Eval81/1(In1)
  M082/2(W2Pos) -> Eval81/2(In2)
  M082/3(W3Pos) -> Eval81/3(In3)
  M082/4(W4Pos) -> Eval81/4(In4)
  Eval81/1(Out1) -> To Workspace81/1
  [in1] -> M083/1(DW1)
  [in2] -> M083/2(DW2)
  [in4] -> M083/3(DW4)
  [in5] -> M083/4(P1W2)
  [in6] -> M083/5(P2W3)
  [in7] -> M083/6(P1W3)
  [in8] -> M083/7(P3W4)
  [in10] -> M083/8(O1)
  [in11] -> M083/9(O2)
  [in12] -> M083/10(O3)
  [in13] -> M083/11(O4)
  [in14] -> M083/12(LD)
  [in15] -> M083/13(CW1C)
  [in16] -> M083/14(CW2C)
  [in17] -> M083/15(CW3C)
  [in18] -> M083/16(CW4C)
  M083/1(W1Pos) -> Eval82/1(In1)
  M083/2(W2Pos) -> Eval82/2(In2)
  M083/3(W3Pos) -> Eval82/3(In3)
  M083/4(W4Pos) -> Eval82/4(In4)
  Eval82/1(Out1) -> To Workspace82/1
  [in1] -> M084/1(DW1)
  [in2] -> M084/2(DW2)
  [in4] -> M084/3(DW4)
  [in5] -> M084/4(P1W2)
  [in6] -> M084/5(P2W3)
  [in7] -> M084/6(P1W3)
  [in8] -> M084/7(P3W4)
  [in10] -> M084/8(O1)
  [in11] -> M084/9(O2)
  [in12] -> M084/10(O3)
  [in13] -> M084/11(O4)
  [in14] -> M084/12(LD)
  [in15] -> M084/13(CW1C)
  [in16] -> M084/14(CW2C)
  [in17] -> M084/15(CW3C)
  [in18] -> M084/16(CW4C)
  M084/1(W1Pos) -> Eval83/1(In1)
  M084/2(W2Pos) -> Eval83/2(In2)
  M084/3(W3Pos) -> Eval83/3(In3)
  M084/4(W4Pos) -> Eval83/4(In4)
  Eval83/1(Out1) -> To Workspace83/1
  [in1] -> M085/1(DW1)
  [in2] -> M085/2(DW2)
  [in4] -> M085/3(DW4)
  [in5] -> M085/4(P1W2)
  [in6] -> M085/5(P2W3)
  [in7] -> M085/6(P1W3)
  [in8] -> M085/7(P3W4)
  [in10] -> M085/8(O1)
  [in11] -> M085/9(O2)
  [in12] -> M085/10(O3)
  [in13] -> M085/11(O4)
  [in14] -> M085/12(LD)
  [in15] -> M085/13(CW1C)
  [in16] -> M085/14(CW2C)
  [in17] -> M085/15(CW3C)
  [in18] -> M085/16(CW4C)
  M085/1(W1Pos) -> Eval84/1(In1)
  M085/2(W2Pos) -> Eval84/2(In2)
  M085/3(W3Pos) -> Eval84/3(In3)
  M085/4(W4Pos) -> Eval84/4(In4)
  Eval84/1(Out1) -> To Workspace84/1
  [in1] -> M086/1(DW1)
  [in2] -> M086/2(DW2)
  [in4] -> M086/3(DW4)
  [in5] -> M086/4(P1W2)
  [in6] -> M086/5(P2W3)
  [in7] -> M086/6(P1W3)
  [in8] -> M086/7(P3W4)
  [in10] -> M086/8(O1)
  [in11] -> M086/9(O2)
  [in12] -> M086/10(O3)
  [in13] -> M086/11(O4)
  [in14] -> M086/12(LD)
  [in15] -> M086/13(CW1C)
  [in16] -> M086/14(CW2C)
  [in17] -> M086/15(CW3C)
  [in18] -> M086/16(CW4C)
  M086/1(W1Pos) -> Eval85/1(In1)
  M086/2(W2Pos) -> Eval85/2(In2)
  M086/3(W3Pos) -> Eval85/3(In3)
  M086/4(W4Pos) -> Eval85/4(In4)
  Eval85/1(Out1) -> To Workspace85/1
  [in1] -> M087/1(DW1)
  [in2] -> M087/2(DW2)
  [in4] -> M087/3(DW4)
  [in5] -> M087/4(P1W2)
  [in6] -> M087/5(P2W3)
  [in7] -> M087/6(P1W3)
  [in8] -> M087/7(P3W4)
  [in10] -> M087/8(O1)
  [in11] -> M087/9(O2)
  [in12] -> M087/10(O3)
  [in13] -> M087/11(O4)
  [in14] -> M087/12(LD)
  [in15] -> M087/13(CW1C)
  [in16] -> M087/14(CW2C)
  [in17] -> M087/15(CW3C)
  [in18] -> M087/16(CW4C)
  M087/1(W1Pos) -> Eval86/1(In1)
  M087/2(W2Pos) -> Eval86/2(In2)
  M087/3(W3Pos) -> Eval86/3(In3)
  M087/4(W4Pos) -> Eval86/4(In4)
  Eval86/1(Out1) -> To Workspace86/1
  [in1] -> M088/1(DW1)
  [in2] -> M088/2(DW2)
  [in4] -> M088/3(DW4)
  [in5] -> M088/4(P1W2)
  [in6] -> M088/5(P2W3)
  [in7] -> M088/6(P1W3)
  [in8] -> M088/7(P3W4)
  [in10] -> M088/8(O1)
  [in11] -> M088/9(O2)
  [in12] -> M088/10(O3)
  [in13] -> M088/11(O4)
  [in14] -> M088/12(LD)
  [in15] -> M088/13(CW1C)
  [in16] -> M088/14(CW2C)
  [in17] -> M088/15(CW3C)
  [in18] -> M088/16(CW4C)
  M088/1(W1Pos) -> Eval87/1(In1)
  M088/2(W2Pos) -> Eval87/2(In2)
  M088/3(W3Pos) -> Eval87/3(In3)
  M088/4(W4Pos) -> Eval87/4(In4)
  Eval87/1(Out1) -> To Workspace87/1
  [in1] -> M089/1(DW1)
  [in2] -> M089/2(DW2)
  [in4] -> M089/3(DW4)
  [in5] -> M089/4(P1W2)
  [in6] -> M089/5(P2W3)
  [in7] -> M089/6(P1W3)
  [in8] -> M089/7(P3W4)
  [in10] -> M089/8(O1)
  [in11] -> M089/9(O2)
  [in12] -> M089/10(O3)
  [in13] -> M089/11(O4)
  [in14] -> M089/12(LD)
  [in15] -> M089/13(CW1C)
  [in16] -> M089/14(CW2C)
  [in17] -> M089/15(CW3C)
  [in18] -> M089/16(CW4C)
  M089/1(W1Pos) -> Eval88/1(In1)
  M089/2(W2Pos) -> Eval88/2(In2)
  M089/3(W3Pos) -> Eval88/3(In3)
  M089/4(W4Pos) -> Eval88/4(In4)
  Eval88/1(Out1) -> To Workspace88/1
  [in1] -> M090/1(DW1)
  [in2] -> M090/2(DW2)
  [in4] -> M090/3(DW4)
  [in5] -> M090/4(P1W2)
  [in6] -> M090/5(P2W3)
  [in7] -> M090/6(P1W3)
  [in8] -> M090/7(P3W4)
  [in10] -> M090/8(O1)
  [in11] -> M090/9(O2)
  [in12] -> M090/10(O3)
  [in13] -> M090/11(O4)
  [in14] -> M090/12(LD)
  [in15] -> M090/13(CW1C)
  [in16] -> M090/14(CW2C)
  [in17] -> M090/15(CW3C)
  [in18] -> M090/16(CW4C)
  M090/1(W1Pos) -> Eval89/1(In1)
  M090/2(W2Pos) -> Eval89/2(In2)
  M090/3(W3Pos) -> Eval89/3(In3)
  M090/4(W4Pos) -> Eval89/4(In4)
  Eval89/1(Out1) -> To Workspace89/1
  [in1] -> M091/1(DW1)
  [in2] -> M091/2(DW2)
  [in4] -> M091/3(DW4)
  [in5] -> M091/4(P1W2)
  [in6] -> M091/5(P2W3)
  [in7] -> M091/6(P1W3)
  [in8] -> M091/7(P3W4)
  [in10] -> M091/8(O1)
  [in11] -> M091/9(O2)
  [in12] -> M091/10(O3)
  [in13] -> M091/11(O4)
  [in14] -> M091/12(LD)
  [in15] -> M091/13(CW1C)
  [in16] -> M091/14(CW2C)
  [in17] -> M091/15(CW3C)
  [in18] -> M091/16(CW4C)
  M091/1(W1Pos) -> Eval90/1(In1)
  M091/2(W2Pos) -> Eval90/2(In2)
  M091/3(W3Pos) -> Eval90/3(In3)
  M091/4(W4Pos) -> Eval90/4(In4)
  Eval90/1(Out1) -> To Workspace90/1
  [in1] -> M092/1(DW1)
  [in2] -> M092/2(DW2)
  [in4] -> M092/3(DW4)
  [in5] -> M092/4(P1W2)
  [in6] -> M092/5(P2W3)
  [in7] -> M092/6(P1W3)
  [in8] -> M092/7(P3W4)
  [in10] -> M092/8(O1)
  [in11] -> M092/9(O2)
  [in12] -> M092/10(O3)
  [in13] -> M092/11(O4)
  [in14] -> M092/12(LD)
  [in15] -> M092/13(CW1C)
  [in16] -> M092/14(CW2C)
  [in17] -> M092/15(CW3C)
  [in18] -> M092/16(CW4C)
  M092/1(W1Pos) -> Eval91/1(In1)
  M092/2(W2Pos) -> Eval91/2(In2)
  M092/3(W3Pos) -> Eval91/3(In3)
  M092/4(W4Pos) -> Eval91/4(In4)
  Eval91/1(Out1) -> To Workspace91/1
  [in1] -> M093/1(DW1)
  [in2] -> M093/2(DW2)
  [in4] -> M093/3(DW4)
  [in5] -> M093/4(P1W2)
  [in6] -> M093/5(P2W3)
  [in7] -> M093/6(P1W3)
  [in8] -> M093/7(P3W4)
  [in10] -> M093/8(O1)
  [in11] -> M093/9(O2)
  [in12] -> M093/10(O3)
  [in13] -> M093/11(O4)
  [in14] -> M093/12(LD)
  [in15] -> M093/13(CW1C)
  [in16] -> M093/14(CW2C)
  [in17] -> M093/15(CW3C)
  [in18] -> M093/16(CW4C)
  M093/1(W1Pos) -> Eval92/1(In1)
  M093/2(W2Pos) -> Eval92/2(In2)
  M093/3(W3Pos) -> Eval92/3(In3)
  M093/4(W4Pos) -> Eval92/4(In4)
  Eval92/1(Out1) -> To Workspace92/1
  [in1] -> M094/1(DW1)
  [in2] -> M094/2(DW2)
  [in4] -> M094/3(DW4)
  [in5] -> M094/4(P1W2)
  [in6] -> M094/5(P2W3)
  [in7] -> M094/6(P1W3)
  [in8] -> M094/7(P3W4)
  [in10] -> M094/8(O1)
  [in11] -> M094/9(O2)
  [in12] -> M094/10(O3)
  [in13] -> M094/11(O4)
  [in14] -> M094/12(LD)
  [in15] -> M094/13(CW1C)
  [in16] -> M094/14(CW2C)
  [in17] -> M094/15(CW3C)
  [in18] -> M094/16(CW4C)
  M094/1(W1Pos) -> Eval93/1(In1)
  M094/2(W2Pos) -> Eval93/2(In2)
  M094/3(W3Pos) -> Eval93/3(In3)
  M094/4(W4Pos) -> Eval93/4(In4)
  Eval93/1(Out1) -> To Workspace93/1
  [in1] -> M095/1(DW1)
  [in2] -> M095/2(DW2)
  [in4] -> M095/3(DW4)
  [in5] -> M095/4(P1W2)
  [in6] -> M095/5(P2W3)
  [in7] -> M095/6(P1W3)
  [in8] -> M095/7(P3W4)
  [in10] -> M095/8(O1)
  [in11] -> M095/9(O2)
  [in12] -> M095/10(O3)
  [in13] -> M095/11(O4)
  [in14] -> M095/12(LD)
  [in15] -> M095/13(CW1C)
  [in16] -> M095/14(CW2C)
  [in17] -> M095/15(CW3C)
  [in18] -> M095/16(CW4C)
  M095/1(W1Pos) -> Eval94/1(In1)
  M095/2(W2Pos) -> Eval94/2(In2)
  M095/3(W3Pos) -> Eval94/3(In3)
  M095/4(W4Pos) -> Eval94/4(In4)
  Eval94/1(Out1) -> To Workspace94/1
  [in1] -> M096/1(DW1)
  [in2] -> M096/2(DW2)
  [in4] -> M096/3(DW4)
  [in5] -> M096/4(P1W2)
  [in6] -> M096/5(P2W3)
  [in7] -> M096/6(P1W3)
  [in8] -> M096/7(P3W4)
  [in10] -> M096/8(O1)
  [in11] -> M096/9(O2)
  [in12] -> M096/10(O3)
  [in13] -> M096/11(O4)
  [in14] -> M096/12(LD)
  [in15] -> M096/13(CW1C)
  [in16] -> M096/14(CW2C)
  [in17] -> M096/15(CW3C)
  [in18] -> M096/16(CW4C)
  M096/1(W1Pos) -> Eval95/1(In1)
  M096/2(W2Pos) -> Eval95/2(In2)
  M096/3(W3Pos) -> Eval95/3(In3)
  M096/4(W4Pos) -> Eval95/4(In4)
  Eval95/1(Out1) -> To Workspace95/1
  [in1] -> M097/1(DW1)
  [in2] -> M097/2(DW2)
  [in4] -> M097/3(DW4)
  [in5] -> M097/4(P1W2)
  [in6] -> M097/5(P2W3)
  [in7] -> M097/6(P1W3)
  [in8] -> M097/7(P3W4)
  [in10] -> M097/8(O1)
  [in11] -> M097/9(O2)
  [in12] -> M097/10(O3)
  [in13] -> M097/11(O4)
  [in14] -> M097/12(LD)
  [in15] -> M097/13(CW1C)
  [in16] -> M097/14(CW2C)
  [in17] -> M097/15(CW3C)
  [in18] -> M097/16(CW4C)
  M097/1(W1Pos) -> Eval96/1(In1)
  M097/2(W2Pos) -> Eval96/2(In2)
  M097/3(W3Pos) -> Eval96/3(In3)
  M097/4(W4Pos) -> Eval96/4(In4)
  Eval96/1(Out1) -> To Workspace96/1
  [in1] -> M098/1(DW1)
  [in2] -> M098/2(DW2)
  [in4] -> M098/3(DW4)
  [in5] -> M098/4(P1W2)
  [in6] -> M098/5(P2W3)
  [in7] -> M098/6(P1W3)
  [in8] -> M098/7(P3W4)
  [in10] -> M098/8(O1)
  [in11] -> M098/9(O2)
  [in12] -> M098/10(O3)
  [in13] -> M098/11(O4)
  [in14] -> M098/12(LD)
  [in15] -> M098/13(CW1C)
  [in16] -> M098/14(CW2C)
  [in17] -> M098/15(CW3C)
  [in18] -> M098/16(CW4C)
  M098/1(W1Pos) -> Eval97/1(In1)
  M098/2(W2Pos) -> Eval97/2(In2)
  M098/3(W3Pos) -> Eval97/3(In3)
  M098/4(W4Pos) -> Eval97/4(In4)
  Eval97/1(Out1) -> To Workspace97/1
  [in1] -> M099/1(DW1)
  [in2] -> M099/2(DW2)
  [in4] -> M099/3(DW4)
  [in5] -> M099/4(P1W2)
  [in6] -> M099/5(P2W3)
  [in7] -> M099/6(P1W3)
  [in8] -> M099/7(P3W4)
  [in10] -> M099/8(O1)
  [in11] -> M099/9(O2)
  [in12] -> M099/10(O3)
  [in13] -> M099/11(O4)
  [in14] -> M099/12(LD)
  [in15] -> M099/13(CW1C)
  [in16] -> M099/14(CW2C)
  [in17] -> M099/15(CW3C)
  [in18] -> M099/16(CW4C)
  M099/1(W1Pos) -> Eval98/1(In1)
  M099/2(W2Pos) -> Eval98/2(In2)
  M099/3(W3Pos) -> Eval98/3(In3)
  M099/4(W4Pos) -> Eval98/4(In4)
  Eval98/1(Out1) -> To Workspace98/1
  [in1] -> M100/1(DW1)
  [in2] -> M100/2(DW2)
  [in4] -> M100/3(DW4)
  [in5] -> M100/4(P1W2)
  [in6] -> M100/5(P2W3)
  [in7] -> M100/6(P1W3)
  [in8] -> M100/7(P3W4)
  [in10] -> M100/8(O1)
  [in11] -> M100/9(O2)
  [in12] -> M100/10(O3)
  [in13] -> M100/11(O4)
  [in14] -> M100/12(LD)
  [in15] -> M100/13(CW1C)
  [in16] -> M100/14(CW2C)
  [in17] -> M100/15(CW3C)
  [in18] -> M100/16(CW4C)
  M100/1(W1Pos) -> Eval99/1(In1)
  M100/2(W2Pos) -> Eval99/2(In2)
  M100/3(W3Pos) -> Eval99/3(In3)
  M100/4(W4Pos) -> Eval99/4(In4)
  Eval99/1(Out1) -> To Workspace99/1
  [in1] -> M101/1(DW1)
  [in2] -> M101/2(DW2)
  [in4] -> M101/3(DW4)
  [in5] -> M101/4(P1W2)
  [in6] -> M101/5(P2W3)
  [in7] -> M101/6(P1W3)
  [in8] -> M101/7(P3W4)
  [in10] -> M101/8(O1)
  [in11] -> M101/9(O2)
  [in12] -> M101/10(O3)
  [in13] -> M101/11(O4)
  [in14] -> M101/12(LD)
  [in15] -> M101/13(CW1C)
  [in16] -> M101/14(CW2C)
  [in17] -> M101/15(CW3C)
  [in18] -> M101/16(CW4C)
  M101/1(W1Pos) -> Eval100/1(In1)
  M101/2(W2Pos) -> Eval100/2(In2)
  M101/3(W3Pos) -> Eval100/3(In3)
  M101/4(W4Pos) -> Eval100/4(In4)
  Eval100/1(Out1) -> To Workspace100/1
  [in1] -> M102/1(DW1)
  [in2] -> M102/2(DW2)
  [in4] -> M102/3(DW4)
  [in5] -> M102/4(P1W2)
  [in6] -> M102/5(P2W3)
  [in7] -> M102/6(P1W3)
  [in8] -> M102/7(P3W4)
  [in10] -> M102/8(O1)
  [in11] -> M102/9(O2)
  [in12] -> M102/10(O3)
  [in13] -> M102/11(O4)
  [in14] -> M102/12(LD)
  [in15] -> M102/13(CW1C)
  [in16] -> M102/14(CW2C)
  [in17] -> M102/15(CW3C)
  [in18] -> M102/16(CW4C)
  M102/1(W1Pos) -> Eval101/1(In1)
  M102/2(W2Pos) -> Eval101/2(In2)
  M102/3(W3Pos) -> Eval101/3(In3)
  M102/4(W4Pos) -> Eval101/4(In4)
  Eval101/1(Out1) -> To Workspace101/1
  [in1] -> M103/1(DW1)
  [in2] -> M103/2(DW2)
  [in4] -> M103/3(DW4)
  [in5] -> M103/4(P1W2)
  [in6] -> M103/5(P2W3)
  [in7] -> M103/6(P1W3)
  [in8] -> M103/7(P3W4)
  [in10] -> M103/8(O1)
  [in11] -> M103/9(O2)
  [in12] -> M103/10(O3)
  [in13] -> M103/11(O4)
  [in14] -> M103/12(LD)
  [in15] -> M103/13(CW1C)
  [in16] -> M103/14(CW2C)
  [in17] -> M103/15(CW3C)
  [in18] -> M103/16(CW4C)
  M103/1(W1Pos) -> Eval102/1(In1)
  M103/2(W2Pos) -> Eval102/2(In2)
  M103/3(W3Pos) -> Eval102/3(In3)
  M103/4(W4Pos) -> Eval102/4(In4)
  Eval102/1(Out1) -> To Workspace102/1
  [in1] -> M104/1(DW1)
  [in2] -> M104/2(DW2)
  [in4] -> M104/3(DW4)
  [in5] -> M104/4(P1W2)
  [in6] -> M104/5(P2W3)
  [in7] -> M104/6(P1W3)
  [in8] -> M104/7(P3W4)
  [in10] -> M104/8(O1)
  [in11] -> M104/9(O2)
  [in12] -> M104/10(O3)
  [in13] -> M104/11(O4)
  [in14] -> M104/12(LD)
  [in15] -> M104/13(CW1C)
  [in16] -> M104/14(CW2C)
  [in17] -> M104/15(CW3C)
  [in18] -> M104/16(CW4C)
  M104/1(W1Pos) -> Eval103/1(In1)
  M104/2(W2Pos) -> Eval103/2(In2)
  M104/3(W3Pos) -> Eval103/3(In3)
  M104/4(W4Pos) -> Eval103/4(In4)
  Eval103/1(Out1) -> To Workspace103/1
  [in1] -> M105/1(DW1)
  [in2] -> M105/2(DW2)
  [in4] -> M105/3(DW4)
  [in5] -> M105/4(P1W2)
  [in6] -> M105/5(P2W3)
  [in7] -> M105/6(P1W3)
  [in8] -> M105/7(P3W4)
  [in10] -> M105/8(O1)
  [in11] -> M105/9(O2)
  [in12] -> M105/10(O3)
  [in13] -> M105/11(O4)
  [in14] -> M105/12(LD)
  [in15] -> M105/13(CW1C)
  [in16] -> M105/14(CW2C)
  [in17] -> M105/15(CW3C)
  [in18] -> M105/16(CW4C)
  M105/1(W1Pos) -> Eval104/1(In1)
  M105/2(W2Pos) -> Eval104/2(In2)
  M105/3(W3Pos) -> Eval104/3(In3)
  M105/4(W4Pos) -> Eval104/4(In4)
  Eval104/1(Out1) -> To Workspace104/1
  [in1] -> M106/1(DW1)
  [in2] -> M106/2(DW2)
  [in4] -> M106/3(DW4)
  [in5] -> M106/4(P1W2)
  [in6] -> M106/5(P2W3)
  [in7] -> M106/6(P1W3)
  [in8] -> M106/7(P3W4)
  [in10] -> M106/8(O1)
  [in11] -> M106/9(O2)
  [in12] -> M106/10(O3)
  [in13] -> M106/11(O4)
  [in14] -> M106/12(LD)
  [in15] -> M106/13(CW1C)
  [in16] -> M106/14(CW2C)
  [in17] -> M106/15(CW3C)
  [in18] -> M106/16(CW4C)
  M106/1(W1Pos) -> Eval105/1(In1)
  M106/2(W2Pos) -> Eval105/2(In2)
  M106/3(W3Pos) -> Eval105/3(In3)
  M106/4(W4Pos) -> Eval105/4(In4)
  Eval105/1(Out1) -> To Workspace105/1
  [in1] -> M107/1(DW1)
  [in2] -> M107/2(DW2)
  [in4] -> M107/3(DW4)
  [in5] -> M107/4(P1W2)
  [in6] -> M107/5(P2W3)
  [in7] -> M107/6(P1W3)
  [in8] -> M107/7(P3W4)
  [in10] -> M107/8(O1)
  [in11] -> M107/9(O2)
  [in12] -> M107/10(O3)
  [in13] -> M107/11(O4)
  [in14] -> M107/12(LD)
  [in15] -> M107/13(CW1C)
  [in16] -> M107/14(CW2C)
  [in17] -> M107/15(CW3C)
  [in18] -> M107/16(CW4C)
  M107/1(W1Pos) -> Eval106/1(In1)
  M107/2(W2Pos) -> Eval106/2(In2)
  M107/3(W3Pos) -> Eval106/3(In3)
  M107/4(W4Pos) -> Eval106/4(In4)
  Eval106/1(Out1) -> To Workspace106/1
  [in1] -> M108/1(DW1)
  [in2] -> M108/2(DW2)
  [in4] -> M108/3(DW4)
  [in5] -> M108/4(P1W2)
  [in6] -> M108/5(P2W3)
  [in7] -> M108/6(P1W3)
  [in8] -> M108/7(P3W4)
  [in10] -> M108/8(O1)
  [in11] -> M108/9(O2)
  [in12] -> M108/10(O3)
  [in13] -> M108/11(O4)
  [in14] -> M108/12(LD)
  [in15] -> M108/13(CW1C)
  [in16] -> M108/14(CW2C)
  [in17] -> M108/15(CW3C)
  [in18] -> M108/16(CW4C)
  M108/1(W1Pos) -> Eval107/1(In1)
  M108/2(W2Pos) -> Eval107/2(In2)
  M108/3(W3Pos) -> Eval107/3(In3)
  M108/4(W4Pos) -> Eval107/4(In4)
  Eval107/1(Out1) -> To Workspace107/1
  [in1] -> M109/1(DW1)
  [in2] -> M109/2(DW2)
  [in4] -> M109/3(DW4)
  [in5] -> M109/4(P1W2)
  [in6] -> M109/5(P2W3)
  [in7] -> M109/6(P1W3)
  [in8] -> M109/7(P3W4)
  [in10] -> M109/8(O1)
  [in11] -> M109/9(O2)
  [in12] -> M109/10(O3)
  [in13] -> M109/11(O4)
  [in14] -> M109/12(LD)
  [in15] -> M109/13(CW1C)
  [in16] -> M109/14(CW2C)
  [in17] -> M109/15(CW3C)
  [in18] -> M109/16(CW4C)
  M109/1(W1Pos) -> Eval108/1(In1)
  M109/2(W2Pos) -> Eval108/2(In2)
  M109/3(W3Pos) -> Eval108/3(In3)
  M109/4(W4Pos) -> Eval108/4(In4)
  Eval108/1(Out1) -> To Workspace108/1
  [in1] -> M110/1(DW1)
  [in2] -> M110/2(DW2)
  [in4] -> M110/3(DW4)
  [in5] -> M110/4(P1W2)
  [in6] -> M110/5(P2W3)
  [in7] -> M110/6(P1W3)
  [in8] -> M110/7(P3W4)
  [in10] -> M110/8(O1)
  [in11] -> M110/9(O2)
  [in12] -> M110/10(O3)
  [in13] -> M110/11(O4)
  [in14] -> M110/12(LD)
  [in15] -> M110/13(CW1C)
  [in16] -> M110/14(CW2C)
  [in17] -> M110/15(CW3C)
  [in18] -> M110/16(CW4C)
  M110/1(W1Pos) -> Eval109/1(In1)
  M110/2(W2Pos) -> Eval109/2(In2)
  M110/3(W3Pos) -> Eval109/3(In3)
  M110/4(W4Pos) -> Eval109/4(In4)
  Eval109/1(Out1) -> To Workspace109/1
  [in1] -> M111/1(DW1)
  [in2] -> M111/2(DW2)
  [in4] -> M111/3(DW4)
  [in5] -> M111/4(P1W2)
  [in6] -> M111/5(P2W3)
  [in7] -> M111/6(P1W3)
  [in8] -> M111/7(P3W4)
  [in10] -> M111/8(O1)
  [in11] -> M111/9(O2)
  [in12] -> M111/10(O3)
  [in13] -> M111/11(O4)
  [in14] -> M111/12(LD)
  [in15] -> M111/13(CW1C)
  [in16] -> M111/14(CW2C)
  [in17] -> M111/15(CW3C)
  [in18] -> M111/16(CW4C)
  M111/1(W1Pos) -> Eval110/1(In1)
  M111/2(W2Pos) -> Eval110/2(In2)
  M111/3(W3Pos) -> Eval110/3(In3)
  M111/4(W4Pos) -> Eval110/4(In4)
  Eval110/1(Out1) -> To Workspace110/1
  [in1] -> M112/1(DW1)
  [in2] -> M112/2(DW2)
  [in4] -> M112/3(DW4)
  [in5] -> M112/4(P1W2)
  [in6] -> M112/5(P2W3)
  [in7] -> M112/6(P1W3)
  [in8] -> M112/7(P3W4)
  [in10] -> M112/8(O1)
  [in11] -> M112/9(O2)
  [in12] -> M112/10(O3)
  [in13] -> M112/11(O4)
  [in14] -> M112/12(LD)
  [in15] -> M112/13(CW1C)
  [in16] -> M112/14(CW2C)
  [in17] -> M112/15(CW3C)
  [in18] -> M112/16(CW4C)
  M112/1(W1Pos) -> Eval111/1(In1)
  M112/2(W2Pos) -> Eval111/2(In2)
  M112/3(W3Pos) -> Eval111/3(In3)
  M112/4(W4Pos) -> Eval111/4(In4)
  Eval111/1(Out1) -> To Workspace111/1
  [in1] -> M113/1(DW1)
  [in2] -> M113/2(DW2)
  [in4] -> M113/3(DW4)
  [in5] -> M113/4(P1W2)
  [in6] -> M113/5(P2W3)
  [in7] -> M113/6(P1W3)
  [in8] -> M113/7(P3W4)
  [in10] -> M113/8(O1)
  [in11] -> M113/9(O2)
  [in12] -> M113/10(O3)
  [in13] -> M113/11(O4)
  [in14] -> M113/12(LD)
  [in15] -> M113/13(CW1C)
  [in16] -> M113/14(CW2C)
  [in17] -> M113/15(CW3C)
  [in18] -> M113/16(CW4C)
  M113/1(W1Pos) -> Eval112/1(In1)
  M113/2(W2Pos) -> Eval112/2(In2)
  M113/3(W3Pos) -> Eval112/3(In3)
  M113/4(W4Pos) -> Eval112/4(In4)
  Eval112/1(Out1) -> To Workspace112/1
  [in1] -> M114/1(DW1)
  [in2] -> M114/2(DW2)
  [in4] -> M114/3(DW4)
  [in5] -> M114/4(P1W2)
  [in6] -> M114/5(P2W3)
  [in7] -> M114/6(P1W3)
  [in8] -> M114/7(P3W4)
  [in10] -> M114/8(O1)
  [in11] -> M114/9(O2)
  [in12] -> M114/10(O3)
  [in13] -> M114/11(O4)
  [in14] -> M114/12(LD)
  [in15] -> M114/13(CW1C)
  [in16] -> M114/14(CW2C)
  [in17] -> M114/15(CW3C)
  [in18] -> M114/16(CW4C)
  M114/1(W1Pos) -> Eval113/1(In1)
  M114/2(W2Pos) -> Eval113/2(In2)
  M114/3(W3Pos) -> Eval113/3(In3)
  M114/4(W4Pos) -> Eval113/4(In4)
  Eval113/1(Out1) -> To Workspace113/1
  [in1] -> M115/1(DW1)
  [in2] -> M115/2(DW2)
  [in4] -> M115/3(DW4)
  [in5] -> M115/4(P1W2)
  [in6] -> M115/5(P2W3)
  [in7] -> M115/6(P1W3)
  [in8] -> M115/7(P3W4)
  [in10] -> M115/8(O1)
  [in11] -> M115/9(O2)
  [in12] -> M115/10(O3)
  [in13] -> M115/11(O4)
  [in14] -> M115/12(LD)
  [in15] -> M115/13(CW1C)
  [in16] -> M115/14(CW2C)
  [in17] -> M115/15(CW3C)
  [in18] -> M115/16(CW4C)
  M115/1(W1Pos) -> Eval114/1(In1)
  M115/2(W2Pos) -> Eval114/2(In2)
  M115/3(W3Pos) -> Eval114/3(In3)
  M115/4(W4Pos) -> Eval114/4(In4)
  Eval114/1(Out1) -> To Workspace114/1
  [in1] -> M116/1(DW1)
  [in2] -> M116/2(DW2)
  [in4] -> M116/3(DW4)
  [in5] -> M116/4(P1W2)
  [in6] -> M116/5(P2W3)
  [in7] -> M116/6(P1W3)
  [in8] -> M116/7(P3W4)
  [in10] -> M116/8(O1)
  [in11] -> M116/9(O2)
  [in12] -> M116/10(O3)
  [in13] -> M116/11(O4)
  [in14] -> M116/12(LD)
  [in15] -> M116/13(CW1C)
  [in16] -> M116/14(CW2C)
  [in17] -> M116/15(CW3C)
  [in18] -> M116/16(CW4C)
  M116/1(W1Pos) -> Eval115/1(In1)
  M116/2(W2Pos) -> Eval115/2(In2)
  M116/3(W3Pos) -> Eval115/3(In3)
  M116/4(W4Pos) -> Eval115/4(In4)
  Eval115/1(Out1) -> To Workspace115/1
  [in1] -> M117/1(DW1)
  [in2] -> M117/2(DW2)
  [in4] -> M117/3(DW4)
  [in5] -> M117/4(P1W2)
  [in6] -> M117/5(P2W3)
  [in7] -> M117/6(P1W3)
  [in8] -> M117/7(P3W4)
  [in10] -> M117/8(O1)
  [in11] -> M117/9(O2)
  [in12] -> M117/10(O3)
  [in13] -> M117/11(O4)
  [in14] -> M117/12(LD)
  [in15] -> M117/13(CW1C)
  [in16] -> M117/14(CW2C)
  [in17] -> M117/15(CW3C)
  [in18] -> M117/16(CW4C)
  M117/1(W1Pos) -> Eval116/1(In1)
  M117/2(W2Pos) -> Eval116/2(In2)
  M117/3(W3Pos) -> Eval116/3(In3)
  M117/4(W4Pos) -> Eval116/4(In4)
  Eval116/1(Out1) -> To Workspace116/1
  [in1] -> M118/1(DW1)
  [in2] -> M118/2(DW2)
  [in4] -> M118/3(DW4)
  [in5] -> M118/4(P1W2)
  [in6] -> M118/5(P2W3)
  [in7] -> M118/6(P1W3)
  [in8] -> M118/7(P3W4)
  [in10] -> M118/8(O1)
  [in11] -> M118/9(O2)
  [in12] -> M118/10(O3)
  [in13] -> M118/11(O4)
  [in14] -> M118/12(LD)
  [in15] -> M118/13(CW1C)
  [in16] -> M118/14(CW2C)
  [in17] -> M118/15(CW3C)
  [in18] -> M118/16(CW4C)
  M118/1(W1Pos) -> Eval117/1(In1)
  M118/2(W2Pos) -> Eval117/2(In2)
  M118/3(W3Pos) -> Eval117/3(In3)
  M118/4(W4Pos) -> Eval117/4(In4)
  Eval117/1(Out1) -> To Workspace117/1
  [in1] -> M119/1(DW1)
  [in2] -> M119/2(DW2)
  [in4] -> M119/3(DW4)
  [in5] -> M119/4(P1W2)
  [in6] -> M119/5(P2W3)
  [in7] -> M119/6(P1W3)
  [in8] -> M119/7(P3W4)
  [in10] -> M119/8(O1)
  [in11] -> M119/9(O2)
  [in12] -> M119/10(O3)
  [in13] -> M119/11(O4)
  [in14] -> M119/12(LD)
  [in15] -> M119/13(CW1C)
  [in16] -> M119/14(CW2C)
  [in17] -> M119/15(CW3C)
  [in18] -> M119/16(CW4C)
  M119/1(W1Pos) -> Eval118/1(In1)
  M119/2(W2Pos) -> Eval118/2(In2)
  M119/3(W3Pos) -> Eval118/3(In3)
  M119/4(W4Pos) -> Eval118/4(In4)
  Eval118/1(Out1) -> To Workspace118/1
  [in1] -> M120/1(DW1)
  [in2] -> M120/2(DW2)
  [in4] -> M120/3(DW4)
  [in5] -> M120/4(P1W2)
  [in6] -> M120/5(P2W3)
  [in7] -> M120/6(P1W3)
  [in8] -> M120/7(P3W4)
  [in10] -> M120/8(O1)
  [in11] -> M120/9(O2)
  [in12] -> M120/10(O3)
  [in13] -> M120/11(O4)
  [in14] -> M120/12(LD)
  [in15] -> M120/13(CW1C)
  [in16] -> M120/14(CW2C)
  [in17] -> M120/15(CW3C)
  [in18] -> M120/16(CW4C)
  M120/1(W1Pos) -> Eval119/1(In1)
  M120/2(W2Pos) -> Eval119/2(In2)
  M120/3(W3Pos) -> Eval119/3(In3)
  M120/4(W4Pos) -> Eval119/4(In4)
  Eval119/1(Out1) -> To Workspace119/1
  [in1] -> M121/1(DW1)
  [in2] -> M121/2(DW2)
  [in4] -> M121/3(DW4)
  [in5] -> M121/4(P1W2)
  [in6] -> M121/5(P2W3)
  [in7] -> M121/6(P1W3)
  [in8] -> M121/7(P3W4)
  [in10] -> M121/8(O1)
  [in11] -> M121/9(O2)
  [in12] -> M121/10(O3)
  [in13] -> M121/11(O4)
  [in14] -> M121/12(LD)
  [in15] -> M121/13(CW1C)
  [in16] -> M121/14(CW2C)
  [in17] -> M121/15(CW3C)
  [in18] -> M121/16(CW4C)
  M121/1(W1Pos) -> Eval120/1(In1)
  M121/2(W2Pos) -> Eval120/2(In2)
  M121/3(W3Pos) -> Eval120/3(In3)
  M121/4(W4Pos) -> Eval120/4(In4)
  Eval120/1(Out1) -> To Workspace120/1
  [in1] -> M122/1(DW1)
  [in2] -> M122/2(DW2)
  [in4] -> M122/3(DW4)
  [in5] -> M122/4(P1W2)
  [in6] -> M122/5(P2W3)
  [in7] -> M122/6(P1W3)
  [in8] -> M122/7(P3W4)
  [in10] -> M122/8(O1)
  [in11] -> M122/9(O2)
  [in12] -> M122/10(O3)
  [in13] -> M122/11(O4)
  [in14] -> M122/12(LD)
  [in15] -> M122/13(CW1C)
  [in16] -> M122/14(CW2C)
  [in17] -> M122/15(CW3C)
  [in18] -> M122/16(CW4C)
  M122/1(W1Pos) -> Eval121/1(In1)
  M122/2(W2Pos) -> Eval121/2(In2)
  M122/3(W3Pos) -> Eval121/3(In3)
  M122/4(W4Pos) -> Eval121/4(In4)
  Eval121/1(Out1) -> To Workspace121/1
  [in1] -> M123/1(DW1)
  [in2] -> M123/2(DW2)
  [in4] -> M123/3(DW4)
  [in5] -> M123/4(P1W2)
  [in6] -> M123/5(P2W3)
  [in7] -> M123/6(P1W3)
  [in8] -> M123/7(P3W4)
  [in10] -> M123/8(O1)
  [in11] -> M123/9(O2)
  [in12] -> M123/10(O3)
  [in13] -> M123/11(O4)
  [in14] -> M123/12(LD)
  [in15] -> M123/13(CW1C)
  [in16] -> M123/14(CW2C)
  [in17] -> M123/15(CW3C)
  [in18] -> M123/16(CW4C)
  M123/1(W1Pos) -> Eval122/1(In1)
  M123/2(W2Pos) -> Eval122/2(In2)
  M123/3(W3Pos) -> Eval122/3(In3)
  M123/4(W4Pos) -> Eval122/4(In4)
  Eval122/1(Out1) -> To Workspace122/1
  [in1] -> M124/1(DW1)
  [in2] -> M124/2(DW2)
  [in4] -> M124/3(DW4)
  [in5] -> M124/4(P1W2)
  [in6] -> M124/5(P2W3)
  [in7] -> M124/6(P1W3)
  [in8] -> M124/7(P3W4)
  [in10] -> M124/8(O1)
  [in11] -> M124/9(O2)
  [in12] -> M124/10(O3)
  [in13] -> M124/11(O4)
  [in14] -> M124/12(LD)
  [in15] -> M124/13(CW1C)
  [in16] -> M124/14(CW2C)
  [in17] -> M124/15(CW3C)
  [in18] -> M124/16(CW4C)
  M124/1(W1Pos) -> Eval123/1(In1)
  M124/2(W2Pos) -> Eval123/2(In2)
  M124/3(W3Pos) -> Eval123/3(In3)
  M124/4(W4Pos) -> Eval123/4(In4)
  Eval123/1(Out1) -> To Workspace123/1
  [in1] -> M125/1(DW1)
  [in2] -> M125/2(DW2)
  [in4] -> M125/3(DW4)
  [in5] -> M125/4(P1W2)
  [in6] -> M125/5(P2W3)
  [in7] -> M125/6(P1W3)
  [in8] -> M125/7(P3W4)
  [in10] -> M125/8(O1)
  [in11] -> M125/9(O2)
  [in12] -> M125/10(O3)
  [in13] -> M125/11(O4)
  [in14] -> M125/12(LD)
  [in15] -> M125/13(CW1C)
  [in16] -> M125/14(CW2C)
  [in17] -> M125/15(CW3C)
  [in18] -> M125/16(CW4C)
  M125/1(W1Pos) -> Eval124/1(In1)
  M125/2(W2Pos) -> Eval124/2(In2)
  M125/3(W3Pos) -> Eval124/3(In3)
  M125/4(W4Pos) -> Eval124/4(In4)
  Eval124/1(Out1) -> To Workspace124/1
  [in1] -> M126/1(DW1)
  [in2] -> M126/2(DW2)
  [in4] -> M126/3(DW4)
  [in5] -> M126/4(P1W2)
  [in6] -> M126/5(P2W3)
  [in7] -> M126/6(P1W3)
  [in8] -> M126/7(P3W4)
  [in10] -> M126/8(O1)
  [in11] -> M126/9(O2)
  [in12] -> M126/10(O3)
  [in13] -> M126/11(O4)
  [in14] -> M126/12(LD)
  [in15] -> M126/13(CW1C)
  [in16] -> M126/14(CW2C)
  [in17] -> M126/15(CW3C)
  [in18] -> M126/16(CW4C)
  M126/1(W1Pos) -> Eval125/1(In1)
  M126/2(W2Pos) -> Eval125/2(In2)
  M126/3(W3Pos) -> Eval125/3(In3)
  M126/4(W4Pos) -> Eval125/4(In4)
  Eval125/1(Out1) -> To Workspace125/1
  [in1] -> M127/1(DW1)
  [in2] -> M127/2(DW2)
  [in4] -> M127/3(DW4)
  [in5] -> M127/4(P1W2)
  [in6] -> M127/5(P2W3)
  [in7] -> M127/6(P1W3)
  [in8] -> M127/7(P3W4)
  [in10] -> M127/8(O1)
  [in11] -> M127/9(O2)
  [in12] -> M127/10(O3)
  [in13] -> M127/11(O4)
  [in14] -> M127/12(LD)
  [in15] -> M127/13(CW1C)
  [in16] -> M127/14(CW2C)
  [in17] -> M127/15(CW3C)
  [in18] -> M127/16(CW4C)
  M127/1(W1Pos) -> Eval126/1(In1)
  M127/2(W2Pos) -> Eval126/2(In2)
  M127/3(W3Pos) -> Eval126/3(In3)
  M127/4(W4Pos) -> Eval126/4(In4)
  Eval126/1(Out1) -> To Workspace126/1
  [in1] -> M128/1(DW1)
  [in2] -> M128/2(DW2)
  [in4] -> M128/3(DW4)
  [in5] -> M128/4(P1W2)
  [in6] -> M128/5(P2W3)
  [in7] -> M128/6(P1W3)
  [in8] -> M128/7(P3W4)
  [in10] -> M128/8(O1)
  [in11] -> M128/9(O2)
  [in12] -> M128/10(O3)
  [in13] -> M128/11(O4)
  [in14] -> M128/12(LD)
  [in15] -> M128/13(CW1C)
  [in16] -> M128/14(CW2C)
  [in17] -> M128/15(CW3C)
  [in18] -> M128/16(CW4C)
  M128/1(W1Pos) -> Eval127/1(In1)
  M128/2(W2Pos) -> Eval127/2(In2)
  M128/3(W3Pos) -> Eval127/3(In3)
  M128/4(W4Pos) -> Eval127/4(In4)
  Eval127/1(Out1) -> To Workspace127/1
  [in1] -> M129/1(DW1)
  [in2] -> M129/2(DW2)
  [in4] -> M129/3(DW4)
  [in5] -> M129/4(P1W2)
  [in6] -> M129/5(P2W3)
  [in7] -> M129/6(P1W3)
  [in8] -> M129/7(P3W4)
  [in10] -> M129/8(O1)
  [in11] -> M129/9(O2)
  [in12] -> M129/10(O3)
  [in13] -> M129/11(O4)
  [in14] -> M129/12(LD)
  [in15] -> M129/13(CW1C)
  [in16] -> M129/14(CW2C)
  [in17] -> M129/15(CW3C)
  [in18] -> M129/16(CW4C)
  M129/1(W1Pos) -> Eval128/1(In1)
  M129/2(W2Pos) -> Eval128/2(In2)
  M129/3(W3Pos) -> Eval128/3(In3)
  M129/4(W4Pos) -> Eval128/4(In4)
  Eval128/1(Out1) -> To Workspace128/1
  [in1] -> M130/1(DW1)
  [in2] -> M130/2(DW2)
  [in4] -> M130/3(DW4)
  [in5] -> M130/4(P1W2)
  [in6] -> M130/5(P2W3)
  [in7] -> M130/6(P1W3)
  [in8] -> M130/7(P3W4)
  [in10] -> M130/8(O1)
  [in11] -> M130/9(O2)
  [in12] -> M130/10(O3)
  [in13] -> M130/11(O4)
  [in14] -> M130/12(LD)
  [in15] -> M130/13(CW1C)
  [in16] -> M130/14(CW2C)
  [in17] -> M130/15(CW3C)
  [in18] -> M130/16(CW4C)
  M130/1(W1Pos) -> Eval129/1(In1)
  M130/2(W2Pos) -> Eval129/2(In2)
  M130/3(W3Pos) -> Eval129/3(In3)
  M130/4(W4Pos) -> Eval129/4(In4)
  Eval129/1(Out1) -> To Workspace129/1
  [in1] -> M131/1(DW1)
  [in2] -> M131/2(DW2)
  [in4] -> M131/3(DW4)
  [in5] -> M131/4(P1W2)
  [in6] -> M131/5(P2W3)
  [in7] -> M131/6(P1W3)
  [in8] -> M131/7(P3W4)
  [in10] -> M131/8(O1)
  [in11] -> M131/9(O2)
  [in12] -> M131/10(O3)
  [in13] -> M131/11(O4)
  [in14] -> M131/12(LD)
  [in15] -> M131/13(CW1C)
  [in16] -> M131/14(CW2C)
  [in17] -> M131/15(CW3C)
  [in18] -> M131/16(CW4C)
  M131/1(W1Pos) -> Eval130/1(In1)
  M131/2(W2Pos) -> Eval130/2(In2)
  M131/3(W3Pos) -> Eval130/3(In3)
  M131/4(W4Pos) -> Eval130/4(In4)
  Eval130/1(Out1) -> To Workspace130/1
  [in1] -> M132/1(DW1)
  [in2] -> M132/2(DW2)
  [in4] -> M132/3(DW4)
  [in5] -> M132/4(P1W2)
  [in6] -> M132/5(P2W3)
  [in7] -> M132/6(P1W3)
  [in8] -> M132/7(P3W4)
  [in10] -> M132/8(O1)
  [in11] -> M132/9(O2)
  [in12] -> M132/10(O3)
  [in13] -> M132/11(O4)
  [in14] -> M132/12(LD)
  [in15] -> M132/13(CW1C)
  [in16] -> M132/14(CW2C)
  [in17] -> M132/15(CW3C)
  [in18] -> M132/16(CW4C)
  M132/1(W1Pos) -> Eval131/1(In1)
  M132/2(W2Pos) -> Eval131/2(In2)
  M132/3(W3Pos) -> Eval131/3(In3)
  M132/4(W4Pos) -> Eval131/4(In4)
  Eval131/1(Out1) -> To Workspace131/1
  [in1] -> M133/1(DW1)
  [in2] -> M133/2(DW2)
  [in4] -> M133/3(DW4)
  [in5] -> M133/4(P1W2)
  [in6] -> M133/5(P2W3)
  [in7] -> M133/6(P1W3)
  [in8] -> M133/7(P3W4)
  [in10] -> M133/8(O1)
  [in11] -> M133/9(O2)
  [in12] -> M133/10(O3)
  [in13] -> M133/11(O4)
  [in14] -> M133/12(LD)
  [in15] -> M133/13(CW1C)
  [in16] -> M133/14(CW2C)
  [in17] -> M133/15(CW3C)
  [in18] -> M133/16(CW4C)
  M133/1(W1Pos) -> Eval132/1(In1)
  M133/2(W2Pos) -> Eval132/2(In2)
  M133/3(W3Pos) -> Eval132/3(In3)
  M133/4(W4Pos) -> Eval132/4(In4)
  Eval132/1(Out1) -> To Workspace132/1
  [in1] -> M134/1(DW1)
  [in2] -> M134/2(DW2)
  [in4] -> M134/3(DW4)
  [in5] -> M134/4(P1W2)
  [in6] -> M134/5(P2W3)
  [in7] -> M134/6(P1W3)
  [in8] -> M134/7(P3W4)
  [in10] -> M134/8(O1)
  [in11] -> M134/9(O2)
  [in12] -> M134/10(O3)
  [in13] -> M134/11(O4)
  [in14] -> M134/12(LD)
  [in15] -> M134/13(CW1C)
  [in16] -> M134/14(CW2C)
  [in17] -> M134/15(CW3C)
  [in18] -> M134/16(CW4C)
  M134/1(W1Pos) -> Eval133/1(In1)
  M134/2(W2Pos) -> Eval133/2(In2)
  M134/3(W3Pos) -> Eval133/3(In3)
  M134/4(W4Pos) -> Eval133/4(In4)
  Eval133/1(Out1) -> To Workspace133/1
  [in1] -> M135/1(DW1)
  [in2] -> M135/2(DW2)
  [in4] -> M135/3(DW4)
  [in5] -> M135/4(P1W2)
  [in6] -> M135/5(P2W3)
  [in7] -> M135/6(P1W3)
  [in8] -> M135/7(P3W4)
  [in10] -> M135/8(O1)
  [in11] -> M135/9(O2)
  [in12] -> M135/10(O3)
  [in13] -> M135/11(O4)
  [in14] -> M135/12(LD)
  [in15] -> M135/13(CW1C)
  [in16] -> M135/14(CW2C)
  [in17] -> M135/15(CW3C)
  [in18] -> M135/16(CW4C)
  M135/1(W1Pos) -> Eval134/1(In1)
  M135/2(W2Pos) -> Eval134/2(In2)
  M135/3(W3Pos) -> Eval134/3(In3)
  M135/4(W4Pos) -> Eval134/4(In4)
  Eval134/1(Out1) -> To Workspace134/1
  [in1] -> M136/1(DW1)
  [in2] -> M136/2(DW2)
  [in4] -> M136/3(DW4)
  [in5] -> M136/4(P1W2)
  [in6] -> M136/5(P2W3)
  [in7] -> M136/6(P1W3)
  [in8] -> M136/7(P3W4)
  [in10] -> M136/8(O1)
  [in11] -> M136/9(O2)
  [in12] -> M136/10(O3)
  [in13] -> M136/11(O4)
  [in14] -> M136/12(LD)
  [in15] -> M136/13(CW1C)
  [in16] -> M136/14(CW2C)
  [in17] -> M136/15(CW3C)
  [in18] -> M136/16(CW4C)
  M136/1(W1Pos) -> Eval135/1(In1)
  M136/2(W2Pos) -> Eval135/2(In2)
  M136/3(W3Pos) -> Eval135/3(In3)
  M136/4(W4Pos) -> Eval135/4(In4)
  Eval135/1(Out1) -> To Workspace135/1
  [in1] -> M137/1(DW1)
  [in2] -> M137/2(DW2)
  [in4] -> M137/3(DW4)
  [in5] -> M137/4(P1W2)
  [in6] -> M137/5(P2W3)
  [in7] -> M137/6(P1W3)
  [in8] -> M137/7(P3W4)
  [in10] -> M137/8(O1)
  [in11] -> M137/9(O2)
  [in12] -> M137/10(O3)
  [in13] -> M137/11(O4)
  [in14] -> M137/12(LD)
  [in15] -> M137/13(CW1C)
  [in16] -> M137/14(CW2C)
  [in17] -> M137/15(CW3C)
  [in18] -> M137/16(CW4C)
  M137/1(W1Pos) -> Eval136/1(In1)
  M137/2(W2Pos) -> Eval136/2(In2)
  M137/3(W3Pos) -> Eval136/3(In3)
  M137/4(W4Pos) -> Eval136/4(In4)
  Eval136/1(Out1) -> To Workspace136/1
  [in1] -> M138/1(DW1)
  [in2] -> M138/2(DW2)
  [in4] -> M138/3(DW4)
  [in5] -> M138/4(P1W2)
  [in6] -> M138/5(P2W3)
  [in7] -> M138/6(P1W3)
  [in8] -> M138/7(P3W4)
  [in10] -> M138/8(O1)
  [in11] -> M138/9(O2)
  [in12] -> M138/10(O3)
  [in13] -> M138/11(O4)
  [in14] -> M138/12(LD)
  [in15] -> M138/13(CW1C)
  [in16] -> M138/14(CW2C)
  [in17] -> M138/15(CW3C)
  [in18] -> M138/16(CW4C)
  M138/1(W1Pos) -> Eval137/1(In1)
  M138/2(W2Pos) -> Eval137/2(In2)
  M138/3(W3Pos) -> Eval137/3(In3)
  M138/4(W4Pos) -> Eval137/4(In4)
  Eval137/1(Out1) -> To Workspace137/1
  [in1] -> M139/1(DW1)
  [in2] -> M139/2(DW2)
  [in4] -> M139/3(DW4)
  [in5] -> M139/4(P1W2)
  [in6] -> M139/5(P2W3)
  [in7] -> M139/6(P1W3)
  [in8] -> M139/7(P3W4)
  [in10] -> M139/8(O1)
  [in11] -> M139/9(O2)
  [in12] -> M139/10(O3)
  [in13] -> M139/11(O4)
  [in14] -> M139/12(LD)
  [in15] -> M139/13(CW1C)
  [in16] -> M139/14(CW2C)
  [in17] -> M139/15(CW3C)
  [in18] -> M139/16(CW4C)
  M139/1(W1Pos) -> Eval138/1(In1)
  M139/2(W2Pos) -> Eval138/2(In2)
  M139/3(W3Pos) -> Eval138/3(In3)
  M139/4(W4Pos) -> Eval138/4(In4)
  Eval138/1(Out1) -> To Workspace138/1
  [in1] -> M140/1(DW1)
  [in2] -> M140/2(DW2)
  [in4] -> M140/3(DW4)
  [in5] -> M140/4(P1W2)
  [in6] -> M140/5(P2W3)
  [in7] -> M140/6(P1W3)
  [in8] -> M140/7(P3W4)
  [in10] -> M140/8(O1)
  [in11] -> M140/9(O2)
  [in12] -> M140/10(O3)
  [in13] -> M140/11(O4)
  [in14] -> M140/12(LD)
  [in15] -> M140/13(CW1C)
  [in16] -> M140/14(CW2C)
  [in17] -> M140/15(CW3C)
  [in18] -> M140/16(CW4C)
  M140/1(W1Pos) -> Eval139/1(In1)
  M140/2(W2Pos) -> Eval139/2(In2)
  M140/3(W3Pos) -> Eval139/3(In3)
  M140/4(W4Pos) -> Eval139/4(In4)
  Eval139/1(Out1) -> To Workspace139/1
  [in1] -> M141/1(DW1)
  [in2] -> M141/2(DW2)
  [in4] -> M141/3(DW4)
  [in5] -> M141/4(P1W2)
  [in6] -> M141/5(P2W3)
  [in7] -> M141/6(P1W3)
  [in8] -> M141/7(P3W4)
  [in10] -> M141/8(O1)
  [in11] -> M141/9(O2)
  [in12] -> M141/10(O3)
  [in13] -> M141/11(O4)
  [in14] -> M141/12(LD)
  [in15] -> M141/13(CW1C)
  [in16] -> M141/14(CW2C)
  [in17] -> M141/15(CW3C)
  [in18] -> M141/16(CW4C)
  M141/1(W1Pos) -> Eval140/1(In1)
  M141/2(W2Pos) -> Eval140/2(In2)
  M141/3(W3Pos) -> Eval140/3(In3)
  M141/4(W4Pos) -> Eval140/4(In4)
  Eval140/1(Out1) -> To Workspace140/1
  [in1] -> M142/1(DW1)
  [in2] -> M142/2(DW2)
  [in4] -> M142/3(DW4)
  [in5] -> M142/4(P1W2)
  [in6] -> M142/5(P2W3)
  [in7] -> M142/6(P1W3)
  [in8] -> M142/7(P3W4)
  [in10] -> M142/8(O1)
  [in11] -> M142/9(O2)
  [in12] -> M142/10(O3)
  [in13] -> M142/11(O4)
  [in14] -> M142/12(LD)
  [in15] -> M142/13(CW1C)
  [in16] -> M142/14(CW2C)
  [in17] -> M142/15(CW3C)
  [in18] -> M142/16(CW4C)
  M142/1(W1Pos) -> Eval141/1(In1)
  M142/2(W2Pos) -> Eval141/2(In2)
  M142/3(W3Pos) -> Eval141/3(In3)
  M142/4(W4Pos) -> Eval141/4(In4)
  Eval141/1(Out1) -> To Workspace141/1
  [in1] -> M143/1(DW1)
  [in2] -> M143/2(DW2)
  [in4] -> M143/3(DW4)
  [in5] -> M143/4(P1W2)
  [in6] -> M143/5(P2W3)
  [in7] -> M143/6(P1W3)
  [in8] -> M143/7(P3W4)
  [in10] -> M143/8(O1)
  [in11] -> M143/9(O2)
  [in12] -> M143/10(O3)
  [in13] -> M143/11(O4)
  [in14] -> M143/12(LD)
  [in15] -> M143/13(CW1C)
  [in16] -> M143/14(CW2C)
  [in17] -> M143/15(CW3C)
  [in18] -> M143/16(CW4C)
  M143/1(W1Pos) -> Eval142/1(In1)
  M143/2(W2Pos) -> Eval142/2(In2)
  M143/3(W3Pos) -> Eval142/3(In3)
  M143/4(W4Pos) -> Eval142/4(In4)
  Eval142/1(Out1) -> To Workspace142/1
  [in1] -> M144/1(DW1)
  [in2] -> M144/2(DW2)
  [in4] -> M144/3(DW4)
  [in5] -> M144/4(P1W2)
  [in6] -> M144/5(P2W3)
  [in7] -> M144/6(P1W3)
  [in8] -> M144/7(P3W4)
  [in10] -> M144/8(O1)
  [in11] -> M144/9(O2)
  [in12] -> M144/10(O3)
  [in13] -> M144/11(O4)
  [in14] -> M144/12(LD)
  [in15] -> M144/13(CW1C)
  [in16] -> M144/14(CW2C)
  [in17] -> M144/15(CW3C)
  [in18] -> M144/16(CW4C)
  M144/1(W1Pos) -> Eval143/1(In1)
  M144/2(W2Pos) -> Eval143/2(In2)
  M144/3(W3Pos) -> Eval143/3(In3)
  M144/4(W4Pos) -> Eval143/4(In4)
  Eval143/1(Out1) -> To Workspace143/1
  [in1] -> M145/1(DW1)
  [in2] -> M145/2(DW2)
  [in4] -> M145/3(DW4)
  [in5] -> M145/4(P1W2)
  [in6] -> M145/5(P2W3)
  [in7] -> M145/6(P1W3)
  [in8] -> M145/7(P3W4)
  [in10] -> M145/8(O1)
  [in11] -> M145/9(O2)
  [in12] -> M145/10(O3)
  [in13] -> M145/11(O4)
  [in14] -> M145/12(LD)
  [in15] -> M145/13(CW1C)
  [in16] -> M145/14(CW2C)
  [in17] -> M145/15(CW3C)
  [in18] -> M145/16(CW4C)
  M145/1(W1Pos) -> Eval144/1(In1)
  M145/2(W2Pos) -> Eval144/2(In2)
  M145/3(W3Pos) -> Eval144/3(In3)
  M145/4(W4Pos) -> Eval144/4(In4)
  Eval144/1(Out1) -> To Workspace144/1
  [in1] -> M146/1(DW1)
  [in2] -> M146/2(DW2)
  [in4] -> M146/3(DW4)
  [in5] -> M146/4(P1W2)
  [in6] -> M146/5(P2W3)
  [in7] -> M146/6(P1W3)
  [in8] -> M146/7(P3W4)
  [in10] -> M146/8(O1)
  [in11] -> M146/9(O2)
  [in12] -> M146/10(O3)
  [in13] -> M146/11(O4)
  [in14] -> M146/12(LD)
  [in15] -> M146/13(CW1C)
  [in16] -> M146/14(CW2C)
  [in17] -> M146/15(CW3C)
  [in18] -> M146/16(CW4C)
  M146/1(W1Pos) -> Eval145/1(In1)
  M146/2(W2Pos) -> Eval145/2(In2)
  M146/3(W3Pos) -> Eval145/3(In3)
  M146/4(W4Pos) -> Eval145/4(In4)
  Eval145/1(Out1) -> To Workspace145/1
  [in1] -> M147/1(DW1)
  [in2] -> M147/2(DW2)
  [in4] -> M147/3(DW4)
  [in5] -> M147/4(P1W2)
  [in6] -> M147/5(P2W3)
  [in7] -> M147/6(P1W3)
  [in8] -> M147/7(P3W4)
  [in10] -> M147/8(O1)
  [in11] -> M147/9(O2)
  [in12] -> M147/10(O3)
  [in13] -> M147/11(O4)
  [in14] -> M147/12(LD)
  [in15] -> M147/13(CW1C)
  [in16] -> M147/14(CW2C)
  [in17] -> M147/15(CW3C)
  [in18] -> M147/16(CW4C)
  M147/1(W1Pos) -> Eval146/1(In1)
  M147/2(W2Pos) -> Eval146/2(In2)
  M147/3(W3Pos) -> Eval146/3(In3)
  M147/4(W4Pos) -> Eval146/4(In4)
  Eval146/1(Out1) -> To Workspace146/1
  [in1] -> M148/1(DW1)
  [in2] -> M148/2(DW2)
  [in4] -> M148/3(DW4)
  [in5] -> M148/4(P1W2)
  [in6] -> M148/5(P2W3)
  [in7] -> M148/6(P1W3)
  [in8] -> M148/7(P3W4)
  [in10] -> M148/8(O1)
  [in11] -> M148/9(O2)
  [in12] -> M148/10(O3)
  [in13] -> M148/11(O4)
  [in14] -> M148/12(LD)
  [in15] -> M148/13(CW1C)
  [in16] -> M148/14(CW2C)
  [in17] -> M148/15(CW3C)
  [in18] -> M148/16(CW4C)
  M148/1(W1Pos) -> Eval147/1(In1)
  M148/2(W2Pos) -> Eval147/2(In2)
  M148/3(W3Pos) -> Eval147/3(In3)
  M148/4(W4Pos) -> Eval147/4(In4)
  Eval147/1(Out1) -> To Workspace147/1
  [in1] -> M149/1(DW1)
  [in2] -> M149/2(DW2)
  [in4] -> M149/3(DW4)
  [in5] -> M149/4(P1W2)
  [in6] -> M149/5(P2W3)
  [in7] -> M149/6(P1W3)
  [in8] -> M149/7(P3W4)
  [in10] -> M149/8(O1)
  [in11] -> M149/9(O2)
  [in12] -> M149/10(O3)
  [in13] -> M149/11(O4)
  [in14] -> M149/12(LD)
  [in15] -> M149/13(CW1C)
  [in16] -> M149/14(CW2C)
  [in17] -> M149/15(CW3C)
  [in18] -> M149/16(CW4C)
  M149/1(W1Pos) -> Eval148/1(In1)
  M149/2(W2Pos) -> Eval148/2(In2)
  M149/3(W3Pos) -> Eval148/3(In3)
  M149/4(W4Pos) -> Eval148/4(In4)
  Eval148/1(Out1) -> To Workspace148/1
  [in1] -> M150/1(DW1)
  [in2] -> M150/2(DW2)
  [in4] -> M150/3(DW4)
  [in5] -> M150/4(P1W2)
  [in6] -> M150/5(P2W3)
  [in7] -> M150/6(P1W3)
  [in8] -> M150/7(P3W4)
  [in10] -> M150/8(O1)
  [in11] -> M150/9(O2)
  [in12] -> M150/10(O3)
  [in13] -> M150/11(O4)
  [in14] -> M150/12(LD)
  [in15] -> M150/13(CW1C)
  [in16] -> M150/14(CW2C)
  [in17] -> M150/15(CW3C)
  [in18] -> M150/16(CW4C)
  M150/1(W1Pos) -> Eval149/1(In1)
  M150/2(W2Pos) -> Eval149/2(In2)
  M150/3(W3Pos) -> Eval149/3(In3)
  M150/4(W4Pos) -> Eval149/4(In4)
  Eval149/1(Out1) -> To Workspace149/1
  [in1] -> M151/1(DW1)
  [in2] -> M151/2(DW2)
  [in4] -> M151/3(DW4)
  [in5] -> M151/4(P1W2)
  [in6] -> M151/5(P2W3)
  [in7] -> M151/6(P1W3)
  [in8] -> M151/7(P3W4)
  [in10] -> M151/8(O1)
  [in11] -> M151/9(O2)
  [in12] -> M151/10(O3)
  [in13] -> M151/11(O4)
  [in14] -> M151/12(LD)
  [in15] -> M151/13(CW1C)
  [in16] -> M151/14(CW2C)
  [in17] -> M151/15(CW3C)
  [in18] -> M151/16(CW4C)
  M151/1(W1Pos) -> Eval150/1(In1)
  M151/2(W2Pos) -> Eval150/2(In2)
  M151/3(W3Pos) -> Eval150/3(In3)
  M151/4(W4Pos) -> Eval150/4(In4)
  Eval150/1(Out1) -> To Workspace150/1
  [in1] -> M152/1(DW1)
  [in2] -> M152/2(DW2)
  [in4] -> M152/3(DW4)
  [in5] -> M152/4(P1W2)
  [in6] -> M152/5(P2W3)
  [in7] -> M152/6(P1W3)
  [in8] -> M152/7(P3W4)
  [in10] -> M152/8(O1)
  [in11] -> M152/9(O2)
  [in12] -> M152/10(O3)
  [in13] -> M152/11(O4)
  [in14] -> M152/12(LD)
  [in15] -> M152/13(CW1C)
  [in16] -> M152/14(CW2C)
  [in17] -> M152/15(CW3C)
  [in18] -> M152/16(CW4C)
  M152/1(W1Pos) -> Eval151/1(In1)
  M152/2(W2Pos) -> Eval151/2(In2)
  M152/3(W3Pos) -> Eval151/3(In3)
  M152/4(W4Pos) -> Eval151/4(In4)
  Eval151/1(Out1) -> To Workspace151/1
  [in1] -> M153/1(DW1)
  [in2] -> M153/2(DW2)
  [in4] -> M153/3(DW4)
  [in5] -> M153/4(P1W2)
  [in6] -> M153/5(P2W3)
  [in7] -> M153/6(P1W3)
  [in8] -> M153/7(P3W4)
  [in10] -> M153/8(O1)
  [in11] -> M153/9(O2)
  [in12] -> M153/10(O3)
  [in13] -> M153/11(O4)
  [in14] -> M153/12(LD)
  [in15] -> M153/13(CW1C)
  [in16] -> M153/14(CW2C)
  [in17] -> M153/15(CW3C)
  [in18] -> M153/16(CW4C)
  M153/1(W1Pos) -> Eval152/1(In1)
  M153/2(W2Pos) -> Eval152/2(In2)
  M153/3(W3Pos) -> Eval152/3(In3)
  M153/4(W4Pos) -> Eval152/4(In4)
  Eval152/1(Out1) -> To Workspace152/1
  [in1] -> M154/1(DW1)
  [in2] -> M154/2(DW2)
  [in4] -> M154/3(DW4)
  [in5] -> M154/4(P1W2)
  [in6] -> M154/5(P2W3)
  [in7] -> M154/6(P1W3)
  [in8] -> M154/7(P3W4)
  [in10] -> M154/8(O1)
  [in11] -> M154/9(O2)
  [in12] -> M154/10(O3)
  [in13] -> M154/11(O4)
  [in14] -> M154/12(LD)
  [in15] -> M154/13(CW1C)
  [in16] -> M154/14(CW2C)
  [in17] -> M154/15(CW3C)
  [in18] -> M154/16(CW4C)
  M154/1(W1Pos) -> Eval153/1(In1)
  M154/2(W2Pos) -> Eval153/2(In2)
  M154/3(W3Pos) -> Eval153/3(In3)
  M154/4(W4Pos) -> Eval153/4(In4)
  Eval153/1(Out1) -> To Workspace153/1
  [in1] -> M155/1(DW1)
  [in2] -> M155/2(DW2)
  [in4] -> M155/3(DW4)
  [in5] -> M155/4(P1W2)
  [in6] -> M155/5(P2W3)
  [in7] -> M155/6(P1W3)
  [in8] -> M155/7(P3W4)
  [in10] -> M155/8(O1)
  [in11] -> M155/9(O2)
  [in12] -> M155/10(O3)
  [in13] -> M155/11(O4)
  [in14] -> M155/12(LD)
  [in15] -> M155/13(CW1C)
  [in16] -> M155/14(CW2C)
  [in17] -> M155/15(CW3C)
  [in18] -> M155/16(CW4C)
  M155/1(W1Pos) -> Eval154/1(In1)
  M155/2(W2Pos) -> Eval154/2(In2)
  M155/3(W3Pos) -> Eval154/3(In3)
  M155/4(W4Pos) -> Eval154/4(In4)
  Eval154/1(Out1) -> To Workspace154/1
  [in1] -> M156/1(DW1)
  [in2] -> M156/2(DW2)
  [in4] -> M156/3(DW4)
  [in5] -> M156/4(P1W2)
  [in6] -> M156/5(P2W3)
  [in7] -> M156/6(P1W3)
  [in8] -> M156/7(P3W4)
  [in10] -> M156/8(O1)
  [in11] -> M156/9(O2)
  [in12] -> M156/10(O3)
  [in13] -> M156/11(O4)
  [in14] -> M156/12(LD)
  [in15] -> M156/13(CW1C)
  [in16] -> M156/14(CW2C)
  [in17] -> M156/15(CW3C)
  [in18] -> M156/16(CW4C)
  M156/1(W1Pos) -> Eval155/1(In1)
  M156/2(W2Pos) -> Eval155/2(In2)
  M156/3(W3Pos) -> Eval155/3(In3)
  M156/4(W4Pos) -> Eval155/4(In4)
  Eval155/1(Out1) -> To Workspace155/1
  [in1] -> M157/1(DW1)
  [in2] -> M157/2(DW2)
  [in4] -> M157/3(DW4)
  [in5] -> M157/4(P1W2)
  [in6] -> M157/5(P2W3)
  [in7] -> M157/6(P1W3)
  [in8] -> M157/7(P3W4)
  [in10] -> M157/8(O1)
  [in11] -> M157/9(O2)
  [in12] -> M157/10(O3)
  [in13] -> M157/11(O4)
  [in14] -> M157/12(LD)
  [in15] -> M157/13(CW1C)
  [in16] -> M157/14(CW2C)
  [in17] -> M157/15(CW3C)
  [in18] -> M157/16(CW4C)
  M157/1(W1Pos) -> Eval156/1(In1)
  M157/2(W2Pos) -> Eval156/2(In2)
  M157/3(W3Pos) -> Eval156/3(In3)
  M157/4(W4Pos) -> Eval156/4(In4)
  Eval156/1(Out1) -> To Workspace156/1
  [in1] -> M158/1(DW1)
  [in2] -> M158/2(DW2)
  [in4] -> M158/3(DW4)
  [in5] -> M158/4(P1W2)
  [in6] -> M158/5(P2W3)
  [in7] -> M158/6(P1W3)
  [in8] -> M158/7(P3W4)
  [in10] -> M158/8(O1)
  [in11] -> M158/9(O2)
  [in12] -> M158/10(O3)
  [in13] -> M158/11(O4)
  [in14] -> M158/12(LD)
  [in15] -> M158/13(CW1C)
  [in16] -> M158/14(CW2C)
  [in17] -> M158/15(CW3C)
  [in18] -> M158/16(CW4C)
  M158/1(W1Pos) -> Eval157/1(In1)
  M158/2(W2Pos) -> Eval157/2(In2)
  M158/3(W3Pos) -> Eval157/3(In3)
  M158/4(W4Pos) -> Eval157/4(In4)
  Eval157/1(Out1) -> To Workspace157/1
  [in1] -> M159/1(DW1)
  [in2] -> M159/2(DW2)
  [in4] -> M159/3(DW4)
  [in5] -> M159/4(P1W2)
  [in6] -> M159/5(P2W3)
  [in7] -> M159/6(P1W3)
  [in8] -> M159/7(P3W4)
  [in10] -> M159/8(O1)
  [in11] -> M159/9(O2)
  [in12] -> M159/10(O3)
  [in13] -> M159/11(O4)
  [in14] -> M159/12(LD)
  [in15] -> M159/13(CW1C)
  [in16] -> M159/14(CW2C)
  [in17] -> M159/15(CW3C)
  [in18] -> M159/16(CW4C)
  M159/1(W1Pos) -> Eval158/1(In1)
  M159/2(W2Pos) -> Eval158/2(In2)
  M159/3(W3Pos) -> Eval158/3(In3)
  M159/4(W4Pos) -> Eval158/4(In4)
  Eval158/1(Out1) -> To Workspace158/1
  [in1] -> M160/1(DW1)
  [in2] -> M160/2(DW2)
  [in4] -> M160/3(DW4)
  [in5] -> M160/4(P1W2)
  [in6] -> M160/5(P2W3)
  [in7] -> M160/6(P1W3)
  [in8] -> M160/7(P3W4)
  [in10] -> M160/8(O1)
  [in11] -> M160/9(O2)
  [in12] -> M160/10(O3)
  [in13] -> M160/11(O4)
  [in14] -> M160/12(LD)
  [in15] -> M160/13(CW1C)
  [in16] -> M160/14(CW2C)
  [in17] -> M160/15(CW3C)
  [in18] -> M160/16(CW4C)
  M160/1(W1Pos) -> Eval159/1(In1)
  M160/2(W2Pos) -> Eval159/2(In2)
  M160/3(W3Pos) -> Eval159/3(In3)
  M160/4(W4Pos) -> Eval159/4(In4)
  Eval159/1(Out1) -> To Workspace159/1
  [in1] -> M161/1(DW1)
  [in2] -> M161/2(DW2)
  [in4] -> M161/3(DW4)
  [in5] -> M161/4(P1W2)
  [in6] -> M161/5(P2W3)
  [in7] -> M161/6(P1W3)
  [in8] -> M161/7(P3W4)
  [in10] -> M161/8(O1)
  [in11] -> M161/9(O2)
  [in12] -> M161/10(O3)
  [in13] -> M161/11(O4)
  [in14] -> M161/12(LD)
  [in15] -> M161/13(CW1C)
  [in16] -> M161/14(CW2C)
  [in17] -> M161/15(CW3C)
  [in18] -> M161/16(CW4C)
  M161/1(W1Pos) -> Eval160/1(In1)
  M161/2(W2Pos) -> Eval160/2(In2)
  M161/3(W3Pos) -> Eval160/3(In3)
  M161/4(W4Pos) -> Eval160/4(In4)
  Eval160/1(Out1) -> To Workspace160/1
  [in1] -> M162/1(DW1)
  [in2] -> M162/2(DW2)
  [in4] -> M162/3(DW4)
  [in5] -> M162/4(P1W2)
  [in6] -> M162/5(P2W3)
  [in7] -> M162/6(P1W3)
  [in8] -> M162/7(P3W4)
  [in10] -> M162/8(O1)
  [in11] -> M162/9(O2)
  [in12] -> M162/10(O3)
  [in13] -> M162/11(O4)
  [in14] -> M162/12(LD)
  [in15] -> M162/13(CW1C)
  [in16] -> M162/14(CW2C)
  [in17] -> M162/15(CW3C)
  [in18] -> M162/16(CW4C)
  M162/1(W1Pos) -> Eval161/1(In1)
  M162/2(W2Pos) -> Eval161/2(In2)
  M162/3(W3Pos) -> Eval161/3(In3)
  M162/4(W4Pos) -> Eval161/4(In4)
  Eval161/1(Out1) -> To Workspace161/1
  [in1] -> M163/1(DW1)
  [in2] -> M163/2(DW2)
  [in4] -> M163/3(DW4)
  [in5] -> M163/4(P1W2)
  [in6] -> M163/5(P2W3)
  [in7] -> M163/6(P1W3)
  [in8] -> M163/7(P3W4)
  [in10] -> M163/8(O1)
  [in11] -> M163/9(O2)
  [in12] -> M163/10(O3)
  [in13] -> M163/11(O4)
  [in14] -> M163/12(LD)
  [in15] -> M163/13(CW1C)
  [in16] -> M163/14(CW2C)
  [in17] -> M163/15(CW3C)
  [in18] -> M163/16(CW4C)
  M163/1(W1Pos) -> Eval162/1(In1)
  M163/2(W2Pos) -> Eval162/2(In2)
  M163/3(W3Pos) -> Eval162/3(In3)
  M163/4(W4Pos) -> Eval162/4(In4)
  Eval162/1(Out1) -> To Workspace162/1
  [in1] -> M164/1(DW1)
  [in2] -> M164/2(DW2)
  [in4] -> M164/3(DW4)
  [in5] -> M164/4(P1W2)
  [in6] -> M164/5(P2W3)
  [in7] -> M164/6(P1W3)
  [in8] -> M164/7(P3W4)
  [in10] -> M164/8(O1)
  [in11] -> M164/9(O2)
  [in12] -> M164/10(O3)
  [in13] -> M164/11(O4)
  [in14] -> M164/12(LD)
  [in15] -> M164/13(CW1C)
  [in16] -> M164/14(CW2C)
  [in17] -> M164/15(CW3C)
  [in18] -> M164/16(CW4C)
  M164/1(W1Pos) -> Eval163/1(In1)
  M164/2(W2Pos) -> Eval163/2(In2)
  M164/3(W3Pos) -> Eval163/3(In3)
  M164/4(W4Pos) -> Eval163/4(In4)
  Eval163/1(Out1) -> To Workspace163/1
  [in1] -> M165/1(DW1)
  [in2] -> M165/2(DW2)
  [in4] -> M165/3(DW4)
  [in5] -> M165/4(P1W2)
  [in6] -> M165/5(P2W3)
  [in7] -> M165/6(P1W3)
  [in8] -> M165/7(P3W4)
  [in10] -> M165/8(O1)
  [in11] -> M165/9(O2)
  [in12] -> M165/10(O3)
  [in13] -> M165/11(O4)
  [in14] -> M165/12(LD)
  [in15] -> M165/13(CW1C)
  [in16] -> M165/14(CW2C)
  [in17] -> M165/15(CW3C)
  [in18] -> M165/16(CW4C)
  M165/1(W1Pos) -> Eval164/1(In1)
  M165/2(W2Pos) -> Eval164/2(In2)
  M165/3(W3Pos) -> Eval164/3(In3)
  M165/4(W4Pos) -> Eval164/4(In4)
  Eval164/1(Out1) -> To Workspace164/1
  [in1] -> M166/1(DW1)
  [in2] -> M166/2(DW2)
  [in4] -> M166/3(DW4)
  [in5] -> M166/4(P1W2)
  [in6] -> M166/5(P2W3)
  [in7] -> M166/6(P1W3)
  [in8] -> M166/7(P3W4)
  [in10] -> M166/8(O1)
  [in11] -> M166/9(O2)
  [in12] -> M166/10(O3)
  [in13] -> M166/11(O4)
  [in14] -> M166/12(LD)
  [in15] -> M166/13(CW1C)
  [in16] -> M166/14(CW2C)
  [in17] -> M166/15(CW3C)
  [in18] -> M166/16(CW4C)
  M166/1(W1Pos) -> Eval165/1(In1)
  M166/2(W2Pos) -> Eval165/2(In2)
  M166/3(W3Pos) -> Eval165/3(In3)
  M166/4(W4Pos) -> Eval165/4(In4)
  Eval165/1(Out1) -> To Workspace165/1
  [in1] -> M167/1(DW1)
  [in2] -> M167/2(DW2)
  [in4] -> M167/3(DW4)
  [in5] -> M167/4(P1W2)
  [in6] -> M167/5(P2W3)
  [in7] -> M167/6(P1W3)
  [in8] -> M167/7(P3W4)
  [in10] -> M167/8(O1)
  [in11] -> M167/9(O2)
  [in12] -> M167/10(O3)
  [in13] -> M167/11(O4)
  [in14] -> M167/12(LD)
  [in15] -> M167/13(CW1C)
  [in16] -> M167/14(CW2C)
  [in17] -> M167/15(CW3C)
  [in18] -> M167/16(CW4C)
  M167/1(W1Pos) -> Eval166/1(In1)
  M167/2(W2Pos) -> Eval166/2(In2)
  M167/3(W3Pos) -> Eval166/3(In3)
  M167/4(W4Pos) -> Eval166/4(In4)
  Eval166/1(Out1) -> To Workspace166/1
  [in1] -> M168/1(DW1)
  [in2] -> M168/2(DW2)
  [in4] -> M168/3(DW4)
  [in5] -> M168/4(P1W2)
  [in6] -> M168/5(P2W3)
  [in7] -> M168/6(P1W3)
  [in8] -> M168/7(P3W4)
  [in10] -> M168/8(O1)
  [in11] -> M168/9(O2)
  [in12] -> M168/10(O3)
  [in13] -> M168/11(O4)
  [in14] -> M168/12(LD)
  [in15] -> M168/13(CW1C)
  [in16] -> M168/14(CW2C)
  [in17] -> M168/15(CW3C)
  [in18] -> M168/16(CW4C)
  M168/1(W1Pos) -> Eval167/1(In1)
  M168/2(W2Pos) -> Eval167/2(In2)
  M168/3(W3Pos) -> Eval167/3(In3)
  M168/4(W4Pos) -> Eval167/4(In4)
  Eval167/1(Out1) -> To Workspace167/1
  [in1] -> M169/1(DW1)
  [in2] -> M169/2(DW2)
  [in4] -> M169/3(DW4)
  [in5] -> M169/4(P1W2)
  [in6] -> M169/5(P2W3)
  [in7] -> M169/6(P1W3)
  [in8] -> M169/7(P3W4)
  [in10] -> M169/8(O1)
  [in11] -> M169/9(O2)
  [in12] -> M169/10(O3)
  [in13] -> M169/11(O4)
  [in14] -> M169/12(LD)
  [in15] -> M169/13(CW1C)
  [in16] -> M169/14(CW2C)
  [in17] -> M169/15(CW3C)
  [in18] -> M169/16(CW4C)
  M169/1(W1Pos) -> Eval168/1(In1)
  M169/2(W2Pos) -> Eval168/2(In2)
  M169/3(W3Pos) -> Eval168/3(In3)
  M169/4(W4Pos) -> Eval168/4(In4)
  Eval168/1(Out1) -> To Workspace168/1
  [in1] -> M170/1(DW1)
  [in2] -> M170/2(DW2)
  [in4] -> M170/3(DW4)
  [in5] -> M170/4(P1W2)
  [in6] -> M170/5(P2W3)
  [in7] -> M170/6(P1W3)
  [in8] -> M170/7(P3W4)
  [in10] -> M170/8(O1)
  [in11] -> M170/9(O2)
  [in12] -> M170/10(O3)
  [in13] -> M170/11(O4)
  [in14] -> M170/12(LD)
  [in15] -> M170/13(CW1C)
  [in16] -> M170/14(CW2C)
  [in17] -> M170/15(CW3C)
  [in18] -> M170/16(CW4C)
  M170/1(W1Pos) -> Eval169/1(In1)
  M170/2(W2Pos) -> Eval169/2(In2)
  M170/3(W3Pos) -> Eval169/3(In3)
  M170/4(W4Pos) -> Eval169/4(In4)
  Eval169/1(Out1) -> To Workspace169/1
  [in1] -> M171/1(DW1)
  [in2] -> M171/2(DW2)
  [in4] -> M171/3(DW4)
  [in5] -> M171/4(P1W2)
  [in6] -> M171/5(P2W3)
  [in7] -> M171/6(P1W3)
  [in8] -> M171/7(P3W4)
  [in10] -> M171/8(O1)
  [in11] -> M171/9(O2)
  [in12] -> M171/10(O3)
  [in13] -> M171/11(O4)
  [in14] -> M171/12(LD)
  [in15] -> M171/13(CW1C)
  [in16] -> M171/14(CW2C)
  [in17] -> M171/15(CW3C)
  [in18] -> M171/16(CW4C)
  M171/1(W1Pos) -> Eval170/1(In1)
  M171/2(W2Pos) -> Eval170/2(In2)
  M171/3(W3Pos) -> Eval170/3(In3)
  M171/4(W4Pos) -> Eval170/4(In4)
  Eval170/1(Out1) -> To Workspace170/1
  [in1] -> M172/1(DW1)
  [in2] -> M172/2(DW2)
  [in4] -> M172/3(DW4)
  [in5] -> M172/4(P1W2)
  [in6] -> M172/5(P2W3)
  [in7] -> M172/6(P1W3)
  [in8] -> M172/7(P3W4)
  [in10] -> M172/8(O1)
  [in11] -> M172/9(O2)
  [in12] -> M172/10(O3)
  [in13] -> M172/11(O4)
  [in14] -> M172/12(LD)
  [in15] -> M172/13(CW1C)
  [in16] -> M172/14(CW2C)
  [in17] -> M172/15(CW3C)
  [in18] -> M172/16(CW4C)
  M172/1(W1Pos) -> Eval171/1(In1)
  M172/2(W2Pos) -> Eval171/2(In2)
  M172/3(W3Pos) -> Eval171/3(In3)
  M172/4(W4Pos) -> Eval171/4(In4)
  Eval171/1(Out1) -> To Workspace171/1
  [in1] -> M173/1(DW1)
  [in2] -> M173/2(DW2)
  [in4] -> M173/3(DW4)
  [in5] -> M173/4(P1W2)
  [in6] -> M173/5(P2W3)
  [in7] -> M173/6(P1W3)
  [in8] -> M173/7(P3W4)
  [in10] -> M173/8(O1)
  [in11] -> M173/9(O2)
  [in12] -> M173/10(O3)
  [in13] -> M173/11(O4)
  [in14] -> M173/12(LD)
  [in15] -> M173/13(CW1C)
  [in16] -> M173/14(CW2C)
  [in17] -> M173/15(CW3C)
  [in18] -> M173/16(CW4C)
  M173/1(W1Pos) -> Eval172/1(In1)
  M173/2(W2Pos) -> Eval172/2(In2)
  M173/3(W3Pos) -> Eval172/3(In3)
  M173/4(W4Pos) -> Eval172/4(In4)
  Eval172/1(Out1) -> To Workspace172/1
  [in1] -> M174/1(DW1)
  [in2] -> M174/2(DW2)
  [in4] -> M174/3(DW4)
  [in5] -> M174/4(P1W2)
  [in6] -> M174/5(P2W3)
  [in7] -> M174/6(P1W3)
  [in8] -> M174/7(P3W4)
  [in10] -> M174/8(O1)
  [in11] -> M174/9(O2)
  [in12] -> M174/10(O3)
  [in13] -> M174/11(O4)
  [in14] -> M174/12(LD)
  [in15] -> M174/13(CW1C)
  [in16] -> M174/14(CW2C)
  [in17] -> M174/15(CW3C)
  [in18] -> M174/16(CW4C)
  M174/1(W1Pos) -> Eval173/1(In1)
  M174/2(W2Pos) -> Eval173/2(In2)
  M174/3(W3Pos) -> Eval173/3(In3)
  M174/4(W4Pos) -> Eval173/4(In4)
  Eval173/1(Out1) -> To Workspace173/1
  Inputs/1(DW1) -> dtc_DW1/1
  dtc_DW1/1 -> CPSUT/1(DW1), [in1]
  Inputs/2(DW2) -> dtc_DW2/1
  dtc_DW2/1 -> CPSUT/2(DW2), [in2]
  Inputs/3(DW4) -> dtc_DW4/1
  dtc_DW4/1 -> CPSUT/3(DW4), [in4]
  Inputs/4(P1W2) -> dtc_P1W2/1
  dtc_P1W2/1 -> CPSUT/4(P1W2), [in5]
  Inputs/5(P2W3) -> dtc_P2W3/1
  dtc_P2W3/1 -> CPSUT/5(P2W3), [in6]
  Inputs/6(P1W3) -> dtc_P1W3/1
  dtc_P1W3/1 -> CPSUT/6(P1W3), [in7]
  Inputs/7(P3W4) -> dtc_P3W4/1
  dtc_P3W4/1 -> CPSUT/7(P3W4), [in8]
  Inputs/8(O1) -> dtc_O1/1
  dtc_O1/1 -> CPSUT/8(O1), [in10]
  Inputs/9(O2) -> dtc_O2/1
  dtc_O2/1 -> CPSUT/9(O2), [in11]
  Inputs/10(O3) -> dtc_O3/1
  dtc_O3/1 -> CPSUT/10(O3), [in12]
  Inputs/11(O4) -> dtc_O4/1
  dtc_O4/1 -> CPSUT/11(O4), [in13]
  Inputs/12(LD) -> dtc_LD/1
  dtc_LD/1 -> CPSUT/12(LD), [in14]
  Inputs/13(CW1C) -> dtc_CW1C/1
  dtc_CW1C/1 -> CPSUT/13(CW1C), [in15]
  Inputs/14(CW2C) -> dtc_CW2C/1
  dtc_CW2C/1 -> CPSUT/14(CW2C), [in16]
  Inputs/15(CW3C) -> dtc_CW3C/1
  dtc_CW3C/1 -> CPSUT/15(CW3C), [in17]
  Inputs/16(CW4C) -> dtc_CW4C/1
  dtc_CW4C/1 -> CPSUT/16(CW4C), [in18]
